simulink library "AEMS_Standard_Library"  (R2016b)
(part 11 of 39)

      settings: AttributesFormatString=%<MaskType>  RTWSystemCode=Nonreusable function  RTWFcnNameOpts=User specified
      mask Help:
      | eval('path_lib=fileparts(which(''AEMS_Standard_Library''));');
      | mskblk=get_param(gcbh,'MaskType');
      | doc_path = [path_lib '\Help\',mskblk,'.pdf'];
      | eval('open(doc_path)');
  AEMS_SUPPLIER_CALL_SEPA_MIN_LPOS : Subsystem  Tag=[LIB]  TreatAsAtomicUnit=on  RTWFcnName=SUPPLIER_CALL_Sepa_min_lpos  mask(AEMS_SUPPLIER_CALL_SEPA_MIN_LPOS){}
      mask help: Minimal separation time between 2 injection, depending on rail pressure and on fuel mass for open and close delays.
      mask init:
      | Thisblk = gcb;
      | model_type_pos = strsplit(Thisblk,'/');%to split all the layer paths in order to get the runnable path
      | runnable_path = [bdroot '/' model_type_pos{2}];%to get the runnable or AIPCALL path
      | trg_port_name = get_param(find_system(runnable_path,'BlockType','TriggerPort'),'Name');%to get the function call trigger name
      | TaskRate = '';%the raster suffix is stored in the parameter 
      | 
      | if ~isempty(trg_port_name)
      |     trg_port_name_spltd = strsplit(trg_port_name{1},'_');%splitting is done in order to get the raster and its type(Sched or Event)
      |     
      |     % checking for rasters of type Sched or Event especially occuring in
      |     % runnables
      |     if ~isempty(regexp(trg_port_name_spltd{1},'^Sched|^Event','once')) 
      |         TaskRate = ['_' regexprep(trg_port_name_spltd{1},'Sched|Event','','once')];
      |         
      |     %checking if the raster is dcmcb and this is applicable only for
      |     %APICALL
      |     elseif ~isempty(regexp([trg_port_name_spltd{1} '_' trg_port_name_spltd{2} '_' ],'^DataServices_DCM_|^RoutineServices_DCM_','once'))||...
      |             ~isempty(regexp(trg_port_name_spltd{1},'^Dcm$','once'))
      |         TaskRate = '_dcmcb';
      |         
      |     %checking if this block is used under the function call trigger
      |     %starting with "Com" and then giving an error message
      |     %this is applicable only for APICALL
      |     elseif ~isempty(regexp(trg_port_name_spltd{1},'^Com$','once'))
      |         msg = sprintf(['\n','The Supplier call block "' Thisblk '" should not be present within APICALLs having function call trigger as "Com"']);
      |         errordlg(msg);
      |         return;
      |     end
      | end
      | 
      | DataName = ['Supplier_Call_Sepa_Po_Lpost' TaskRate];%the variable name that should be given to DataStoreRead block 
      | set_param([Thisblk '/Data Store Read'],'DataStoreName',DataName);%Setting the DataStoreName of DataStoreRead block
      | 
      | %other settings done to this variable name
      | structVxx=Simulink.Signal;
      | structVxx.Dimensions=1;
      | structVxx.DimensionsMode='Fixed';
      | structVxx.DataType='single';
      | structVxx.Complexity='real';
      | structVxx.SamplingMode='Sample based';
      | structVxx.SampleTime=-1;
      | assignin('base',DataName,structVxx);
      settings: AttributesFormatString=%<MaskType>  RTWSystemCode=Nonreusable function  RTWFcnNameOpts=User specified
      mask Help:
      | eval('path_lib=fileparts(which(''AEMS_Standard_Library''));');
      | mskblk=get_param(gcbh,'MaskType');
      | doc_path = [path_lib '\Help\',mskblk,'.pdf'];
      | eval('open(doc_path)');
  AEMS_SUPPLIER_CALL_SEPA_MIN_LPOS2_2SL : Subsystem  Tag=[LIB]  TreatAsAtomicUnit=on  RTWFcnName=SUPPLIER_CALL_Sepa_min_lpos2_2sl  mask(AEMS_SUPPLIER_CALL_SEPA_MIN_LPOS2_2SL){}
      mask help: Minimal separation time between 2 injection, depending on rail pressure and on fuel mass for open and close delays.
      mask init:
      | Thisblk = gcb;
      | model_type_pos = strsplit(Thisblk,'/');%to split all the layer paths in order to get the runnable path
      | runnable_path = [bdroot '/' model_type_pos{2}];%to get the runnable or AIPCALL path
      | trg_port_name = get_param(find_system(runnable_path,'BlockType','TriggerPort'),'Name');%to get the function call trigger name
      | TaskRate = '';%the raster suffix is stored in the parameter 
      | 
      | if ~isempty(trg_port_name)
      |     trg_port_name_spltd = strsplit(trg_port_name{1},'_');%splitting is done in order to get the raster and its type(Sched or Event)
      |     
      |     % checking for rasters of type Sched or Event especially occuring in
      |     % runnables
      |     if ~isempty(regexp(trg_port_name_spltd{1},'^Sched|^Event','once')) 
      |         TaskRate = ['_' regexprep(trg_port_name_spltd{1},'Sched|Event','','once')];
      |         
      |     %checking if the raster is dcmcb and this is applicable only for
      |     %APICALL
      |     elseif ~isempty(regexp([trg_port_name_spltd{1} '_' trg_port_name_spltd{2} '_' ],'^DataServices_DCM_|^RoutineServices_DCM_','once'))||...
      |             ~isempty(regexp(trg_port_name_spltd{1},'^Dcm$','once'))
      |         TaskRate = '_dcmcb';
      |         
      |     %checking if this block is used under the function call trigger
      |     %starting with "Com" and then giving an error message
      |     %this is applicable only for APICALL
      |     elseif ~isempty(regexp(trg_port_name_spltd{1},'^Com$','once'))
      |         msg = sprintf(['\n','The Supplier call block "' Thisblk '" should not be present within APICALLs having function call trigger as "Com"']);
      |         errordlg(msg);
      |         return;
      |     end
      | end
      | 
      | DataName = ['Supplier_Call_Sepa_Lpost1_Lpost2' TaskRate];%the variable name that should be given to DataStoreRead block 
      | set_param([Thisblk '/Data Store Read'],'DataStoreName',DataName);%Setting the DataStoreName of DataStoreRead block
      | 
      | %other settings done to this variable name
      | structVxx=Simulink.Signal;
      | structVxx.Dimensions=1;
      | structVxx.DimensionsMode='Fixed';
      | structVxx.DataType='single';
      | structVxx.Complexity='real';
      | structVxx.SamplingMode='Sample based';
      | structVxx.SampleTime=-1;
      | assignin('base',DataName,structVxx);
      settings: AttributesFormatString=%<MaskType>  RTWSystemCode=Nonreusable function  RTWFcnNameOpts=User specified
      mask Help:
      | eval('path_lib=fileparts(which(''AEMS_Standard_Library''));');
      | mskblk=get_param(gcbh,'MaskType');
      | doc_path = [path_lib '\Help\',mskblk,'.pdf'];
      | eval('open(doc_path)');
  AEMS_SUPPLIER_CALL_SEPA_MIN_LPOS2_3SL : Subsystem  Tag=[LIB]  TreatAsAtomicUnit=on  RTWFcnName=SUPPLIER_CALL_Sepa_min_lpos2_3sl  mask(AEMS_SUPPLIER_CALL_SEPA_MIN_LPOS2_3SL){}
      mask help: Minimal separation time between 2 injection, depending on rail pressure and on fuel mass for open and close delays.
      mask init: same as AEMS_Standard_Library/SPECIFIC/AEMS_SUPPLIER_CALL_SEPA_MIN_LPOS2_2SL
      settings: AttributesFormatString=%<MaskType>  RTWSystemCode=Nonreusable function  RTWFcnNameOpts=User specified
      mask Help:
      | eval('path_lib=fileparts(which(''AEMS_Standard_Library''));');
      | mskblk=get_param(gcbh,'MaskType');
      | doc_path = [path_lib '\Help\',mskblk,'.pdf'];
      | eval('open(doc_path)');
  AEMS_SUPPLIER_CALL_SEPA_MIN_LPOS2_4SL : Subsystem  Tag=[LIB]  TreatAsAtomicUnit=on  RTWFcnName=SUPPLIER_CALL_Sepa_min_lpos2_4sl  mask(AEMS_SUPPLIER_CALL_SEPA_MIN_LPOS2_4SL){}
      mask help: Minimal separation time between 2 injection, depending on rail pressure and on fuel mass for open and close delays.
      mask init: same as AEMS_Standard_Library/SPECIFIC/AEMS_SUPPLIER_CALL_SEPA_MIN_LPOS2_2SL
      settings: AttributesFormatString=%<MaskType>  RTWSystemCode=Nonreusable function  RTWFcnNameOpts=User specified
      mask Help:
      | eval('path_lib=fileparts(which(''AEMS_Standard_Library''));');
      | mskblk=get_param(gcbh,'MaskType');
      | doc_path = [path_lib '\Help\',mskblk,'.pdf'];
      | eval('open(doc_path)');
  AEMS_SUPPLIER_CALL_SEPA_MIN_LPOS3_3SL : Subsystem  Tag=[LIB]  TreatAsAtomicUnit=on  RTWFcnName=SUPPLIER_CALL_Sepa_min_lpos3_3sl  mask(AEMS_SUPPLIER_CALL_SEPA_MIN_LPOS3_3SL){}
      mask help: Minimal separation time between 2 injection, depending on rail pressure and on fuel mass for open and close delays.
      mask init: same as AEMS_Standard_Library/SPECIFIC/AEMS_SUPPLIER_CALL_SEPA_MIN_LPOS2_2SL
      settings: AttributesFormatString=%<MaskType>  RTWSystemCode=Nonreusable function  RTWFcnNameOpts=User specified
      mask Help:
      | eval('path_lib=fileparts(which(''AEMS_Standard_Library''));');
      | mskblk=get_param(gcbh,'MaskType');
      | doc_path = [path_lib '\Help\',mskblk,'.pdf'];
      | eval('open(doc_path)');
  AEMS_SUPPLIER_CALL_SEPA_MIN_LPOS3_4SL : Subsystem  Tag=[LIB]  TreatAsAtomicUnit=on  RTWFcnName=SUPPLIER_CALL_Sepa_min_lpos3_4sl  mask(AEMS_SUPPLIER_CALL_SEPA_MIN_LPOS3_4SL){}
      mask help: Minimal separation time between 2 injection, depending on rail pressure and on fuel mass for open and close delays.
      mask init: same as AEMS_Standard_Library/SPECIFIC/AEMS_SUPPLIER_CALL_SEPA_MIN_LPOS2_2SL
      settings: AttributesFormatString=%<MaskType>  RTWSystemCode=Nonreusable function  RTWFcnNameOpts=User specified
      mask Help:
      | eval('path_lib=fileparts(which(''AEMS_Standard_Library''));');
      | mskblk=get_param(gcbh,'MaskType');
      | doc_path = [path_lib '\Help\',mskblk,'.pdf'];
      | eval('open(doc_path)');
  AEMS_SUPPLIER_CALL_SEPA_MIN_LPOS4_4SL : Subsystem  Tag=[LIB]  TreatAsAtomicUnit=on  RTWFcnName=SUPPLIER_CALL_Sepa_min_lpos4_4sl  mask(AEMS_SUPPLIER_CALL_SEPA_MIN_LPOS4_4SL){}
      mask help: Minimal separation time between 2 injection, depending on rail pressure and on fuel mass for open and close delays.
      mask init: same as AEMS_Standard_Library/SPECIFIC/AEMS_SUPPLIER_CALL_SEPA_MIN_LPOS2_2SL
      settings: AttributesFormatString=%<MaskType>  RTWSystemCode=Nonreusable function  RTWFcnNameOpts=User specified
      mask Help:
      | eval('path_lib=fileparts(which(''AEMS_Standard_Library''));');
      | mskblk=get_param(gcbh,'MaskType');
      | doc_path = [path_lib '\Help\',mskblk,'.pdf'];
      | eval('open(doc_path)');
  AEMS_SUPPLIER_CALL_SEPA_MIN_NXT_CYL : Subsystem  Tag=[LIB]  TreatAsAtomicUnit=on  RTWFcnName=SUPPLIER_CALL_Sepa_min_nxt_cyl  mask(AEMS_SUPPLIER_CALL_SEPA_MIN_NXT_CYL){}
      mask help: Minimal separation time between 2 injection, depending on rail pressure and on fuel mass for open and close delays.
      mask init:
      | Thisblk = gcb;
      | model_type_pos = strsplit(Thisblk,'/');%to split all the layer paths in order to get the runnable path
      | runnable_path = [bdroot '/' model_type_pos{2}];%to get the runnable or AIPCALL path
      | trg_port_name = get_param(find_system(runnable_path,'BlockType','TriggerPort'),'Name');%to get the function call trigger name
      | TaskRate = '';%the raster suffix is stored in the parameter 
      | 
      | if ~isempty(trg_port_name)
      |     trg_port_name_spltd = strsplit(trg_port_name{1},'_');%splitting is done in order to get the raster and its type(Sched or Event)
      |     
      |     % checking for rasters of type Sched or Event especially occuring in
      |     % runnables
      |     if ~isempty(regexp(trg_port_name_spltd{1},'^Sched|^Event','once')) 
      |         TaskRate = ['_' regexprep(trg_port_name_spltd{1},'Sched|Event','','once')];
      |         
      |     %checking if the raster is dcmcb and this is applicable only for
      |     %APICALL
      |     elseif ~isempty(regexp([trg_port_name_spltd{1} '_' trg_port_name_spltd{2} '_' ],'^DataServices_DCM_|^RoutineServices_DCM_','once'))||...
      |             ~isempty(regexp(trg_port_name_spltd{1},'^Dcm$','once'))
      |         TaskRate = '_dcmcb';
      |         
      |     %checking if this block is used under the function call trigger
      |     %starting with "Com" and then giving an error message
      |     %this is applicable only for APICALL
      |     elseif ~isempty(regexp(trg_port_name_spltd{1},'^Com$','once'))
      |         msg = sprintf(['\n','The Supplier call block "' Thisblk '" should not be present within APICALLs having function call trigger as "Com"']);
      |         errordlg(msg);
      |         return;
      |     end
      | end
      | 
      | DataName = ['Supplier_Call_Sepa_Lpost_Pinj' TaskRate];%the variable name that should be given to DataStoreRead block 
      | set_param([Thisblk '/Data Store Read'],'DataStoreName',DataName);%Setting the DataStoreName of DataStoreRead block
      | 
      | %other settings done to this variable name
      | structVxx=Simulink.Signal;
      | structVxx.Dimensions=1;
      | structVxx.DimensionsMode='Fixed';
      | structVxx.DataType='single';
      | structVxx.Complexity='real';
      | structVxx.SamplingMode='Sample based';
      | structVxx.SampleTime=-1;
      | assignin('base',DataName,structVxx);
      settings: AttributesFormatString=%<MaskType>  RTWSystemCode=Nonreusable function  RTWFcnNameOpts=User specified
      mask Help:
      | eval('path_lib=fileparts(which(''AEMS_Standard_Library''));');
      | mskblk=get_param(gcbh,'MaskType');
      | doc_path = [path_lib '\Help\',mskblk,'.pdf'];
      | eval('open(doc_path)');
  AEMS_SUPPLIER_CALL_SEPA_MIN_NXT_CYL_LPOST2 : Subsystem  Tag=[LIB]  TreatAsAtomicUnit=on  RTWFcnName=SUPPLIER_CALL_Sepa_min_nxt_cyl_lpost2  mask(AEMS_SUPPLIER_CALL_SEPA_MIN_NXT_CYL_LPOST2){}
      mask help: Minimal separation time between 2 injection, depending on rail pressure and on fuel mass for open and close delays.
      mask init: same as AEMS_Standard_Library/SPECIFIC/AEMS_SUPPLIER_CALL_SEPA_MIN_NXT_CYL
      settings: AttributesFormatString=%<MaskType>  RTWSystemCode=Nonreusable function  RTWFcnNameOpts=User specified
      mask Help:
      | eval('path_lib=fileparts(which(''AEMS_Standard_Library''));');
      | mskblk=get_param(gcbh,'MaskType');
      | doc_path = [path_lib '\Help\',mskblk,'.pdf'];
      | eval('open(doc_path)');
  AEMS_SUPPLIER_CALL_SEPA_MIN_NXT_CYL_LPOST3 : Subsystem  Tag=[LIB]  TreatAsAtomicUnit=on  RTWFcnName=SUPPLIER_CALL_Sepa_min_nxt_cyl_lpost3  mask(AEMS_SUPPLIER_CALL_SEPA_MIN_NXT_CYL_LPOST3){}
      mask help: Minimal separation time between 2 injection, depending on rail pressure and on fuel mass for open and close delays.
      mask init: same as AEMS_Standard_Library/SPECIFIC/AEMS_SUPPLIER_CALL_SEPA_MIN_NXT_CYL
      settings: AttributesFormatString=%<MaskType>  RTWSystemCode=Nonreusable function  RTWFcnNameOpts=User specified
      mask Help:
      | eval('path_lib=fileparts(which(''AEMS_Standard_Library''));');
      | mskblk=get_param(gcbh,'MaskType');
      | doc_path = [path_lib '\Help\',mskblk,'.pdf'];
      | eval('open(doc_path)');
  AEMS_SUPPLIER_CALL_SEPA_MIN_NXT_CYL_LPOST4 : Subsystem  Tag=[LIB]  TreatAsAtomicUnit=on  RTWFcnName=SUPPLIER_CALL_Sepa_min_nxt_cyl_lpost4  mask(AEMS_SUPPLIER_CALL_SEPA_MIN_NXT_CYL_LPOST4){}
      mask help: Minimal separation time between 2 injection, depending on rail pressure and on fuel mass for open and close delays.
      mask init: same as AEMS_Standard_Library/SPECIFIC/AEMS_SUPPLIER_CALL_SEPA_MIN_NXT_CYL
      settings: AttributesFormatString=%<MaskType>  RTWSystemCode=Nonreusable function  RTWFcnNameOpts=User specified
      mask Help:
      | eval('path_lib=fileparts(which(''AEMS_Standard_Library''));');
      | mskblk=get_param(gcbh,'MaskType');
      | doc_path = [path_lib '\Help\',mskblk,'.pdf'];
      | eval('open(doc_path)');
  AEMS_SUPPLIER_CALL_SEPA_MIN_PINJ1 : Subsystem  Tag=[LIB]  TreatAsAtomicUnit=on  RTWFcnName=SUPPLIER_CALL_Sepa_min_pinj1  mask(AEMS_SUPPLIER_CALL_SEPA_MIN_PINJ1){}
      mask help: Minimal separation time between 2 injection, depending on rail pressure and on fuel mass for open and close delays.
      mask init:
      | Thisblk = gcb;
      | model_type_pos = strsplit(Thisblk,'/');%to split all the layer paths in order to get the runnable path
      | runnable_path = [bdroot '/' model_type_pos{2}];%to get the runnable or AIPCALL path
      | trg_port_name = get_param(find_system(runnable_path,'BlockType','TriggerPort'),'Name');%to get the function call trigger name
      | TaskRate = '';%the raster suffix is stored in the parameter 
      | 
      | if ~isempty(trg_port_name)
      |     trg_port_name_spltd = strsplit(trg_port_name{1},'_');%splitting is done in order to get the raster and its type(Sched or Event)
      |     
      |     % checking for rasters of type Sched or Event especially occuring in
      |     % runnables
      |     if ~isempty(regexp(trg_port_name_spltd{1},'^Sched|^Event','once')) 
      |         TaskRate = ['_' regexprep(trg_port_name_spltd{1},'Sched|Event','','once')];
      |         
      |     %checking if the raster is dcmcb and this is applicable only for
      |     %APICALL
      |     elseif ~isempty(regexp([trg_port_name_spltd{1} '_' trg_port_name_spltd{2} '_' ],'^DataServices_DCM_|^RoutineServices_DCM_','once'))||...
      |             ~isempty(regexp(trg_port_name_spltd{1},'^Dcm$','once'))
      |         TaskRate = '_dcmcb';
      |         
      |     %checking if this block is used under the function call trigger
      |     %starting with "Com" and then giving an error message
      |     %this is applicable only for APICALL
      |     elseif ~isempty(regexp(trg_port_name_spltd{1},'^Com$','once'))
      |         msg = sprintf(['\n','The Supplier call block "' Thisblk '" should not be present within APICALLs having function call trigger as "Com"']);
      |         errordlg(msg);
      |         return;
      |     end
      | end
      | 
      | DataName = ['Supplier_Call_Sepa_P1_P2' TaskRate];%the variable name that should be given to DataStoreRead block 
      | set_param([Thisblk '/Data Store Read'],'DataStoreName',DataName);%Setting the DataStoreName of DataStoreRead block
      | 
      | %other settings done to this variable name
      | structVxx=Simulink.Signal;
      | structVxx.Dimensions=1;
      | structVxx.DimensionsMode='Fixed';
      | structVxx.DataType='single';
      | structVxx.Complexity='real';
      | structVxx.SamplingMode='Sample based';
      | structVxx.SampleTime=-1;
      | assignin('base',DataName,structVxx);
      settings: AttributesFormatString=%<MaskType>  RTWSystemCode=Nonreusable function  RTWFcnNameOpts=User specified
      mask Help:
      | eval('path_lib=fileparts(which(''AEMS_Standard_Library''));');
      | mskblk=get_param(gcbh,'MaskType');
      | doc_path = [path_lib '\Help\',mskblk,'.pdf'];
      | eval('open(doc_path)');
  AEMS_SUPPLIER_CALL_SEPA_MIN_PINJ2 : Subsystem  Tag=[LIB]  TreatAsAtomicUnit=on  RTWFcnName=SUPPLIER_CALL_Sepa_min_pinj2  mask(AEMS_SUPPLIER_CALL_SEPA_MIN_PINJ2){}
      mask help: Minimal separation time between 2 injection, depending on rail pressure and on fuel mass for open and close delays.
      mask init:
      | Thisblk = gcb;
      | model_type_pos = strsplit(Thisblk,'/');%to split all the layer paths in order to get the runnable path
      | runnable_path = [bdroot '/' model_type_pos{2}];%to get the runnable or AIPCALL path
      | trg_port_name = get_param(find_system(runnable_path,'BlockType','TriggerPort'),'Name');%to get the function call trigger name
      | TaskRate = '';%the raster suffix is stored in the parameter 
      | 
      | if ~isempty(trg_port_name)
      |     trg_port_name_spltd = strsplit(trg_port_name{1},'_');%splitting is done in order to get the raster and its type(Sched or Event)
      |     
      |     % checking for rasters of type Sched or Event especially occuring in
      |     % runnables
      |     if ~isempty(regexp(trg_port_name_spltd{1},'^Sched|^Event','once')) 
      |         TaskRate = ['_' regexprep(trg_port_name_spltd{1},'Sched|Event','','once')];
      |         
      |     %checking if the raster is dcmcb and this is applicable only for
      |     %APICALL
      |     elseif ~isempty(regexp([trg_port_name_spltd{1} '_' trg_port_name_spltd{2} '_' ],'^DataServices_DCM_|^RoutineServices_DCM_','once'))||...
      |             ~isempty(regexp(trg_port_name_spltd{1},'^Dcm$','once'))
      |         TaskRate = '_dcmcb';
      |         
      |     %checking if this block is used under the function call trigger
      |     %starting with "Com" and then giving an error message
      |     %this is applicable only for APICALL
      |     elseif ~isempty(regexp(trg_port_name_spltd{1},'^Com$','once'))
      |         msg = sprintf(['\n','The Supplier call block "' Thisblk '" should not be present within APICALLs having function call trigger as "Com"']);
      |         errordlg(msg);
      |         return;
      |     end
      | end
      | 
      | DataName = ['Supplier_Call_Sepa_P2_P3' TaskRate];%the variable name that should be given to DataStoreRead block 
      | set_param([Thisblk '/Data Store Read'],'DataStoreName',DataName);%Setting the DataStoreName of DataStoreRead block
      | 
      | %other settings done to this variable name
      | structVxx=Simulink.Signal;
      | structVxx.Dimensions=1;
      | structVxx.DimensionsMode='Fixed';
      | structVxx.DataType='single';
      | structVxx.Complexity='real';
      | structVxx.SamplingMode='Sample based';
      | structVxx.SampleTime=-1;
      | assignin('base',DataName,structVxx);
      settings: AttributesFormatString=%<MaskType>  RTWSystemCode=Nonreusable function  RTWFcnNameOpts=User specified
      mask Help:
      | eval('path_lib=fileparts(which(''AEMS_Standard_Library''));');
      | mskblk=get_param(gcbh,'MaskType');
      | doc_path = [path_lib '\Help\',mskblk,'.pdf'];
      | eval('open(doc_path)');
  AEMS_SUPPLIER_CALL_SEPA_MIN_PINJ3 : Subsystem  Tag=[LIB]  TreatAsAtomicUnit=on  RTWFcnName=SUPPLIER_CALL_Sepa_min_pinj3  mask(AEMS_SUPPLIER_CALL_SEPA_MIN_PINJ3){}
      mask help: Minimal separation time between 2 injection, depending on rail pressure and on fuel mass for open and close delays.
      mask init:
      | Thisblk = gcb;
      | model_type_pos = strsplit(Thisblk,'/');%to split all the layer paths in order to get the runnable path
      | runnable_path = [bdroot '/' model_type_pos{2}];%to get the runnable or AIPCALL path
      | trg_port_name = get_param(find_system(runnable_path,'BlockType','TriggerPort'),'Name');%to get the function call trigger name
      | TaskRate = '';%the raster suffix is stored in the parameter 
      | 
      | if ~isempty(trg_port_name)
      |     trg_port_name_spltd = strsplit(trg_port_name{1},'_');%splitting is done in order to get the raster and its type(Sched or Event)
      |     
      |     % checking for rasters of type Sched or Event especially occuring in
      |     % runnables
      |     if ~isempty(regexp(trg_port_name_spltd{1},'^Sched|^Event','once')) 
      |         TaskRate = ['_' regexprep(trg_port_name_spltd{1},'Sched|Event','','once')];
      |         
      |     %checking if the raster is dcmcb and this is applicable only for
      |     %APICALL
      |     elseif ~isempty(regexp([trg_port_name_spltd{1} '_' trg_port_name_spltd{2} '_' ],'^DataServices_DCM_|^RoutineServices_DCM_','once'))||...
      |             ~isempty(regexp(trg_port_name_spltd{1},'^Dcm$','once'))
      |         TaskRate = '_dcmcb';
      |         
      |     %checking if this block is used under the function call trigger
      |     %starting with "Com" and then giving an error message
      |     %this is applicable only for APICALL
      |     elseif ~isempty(regexp(trg_port_name_spltd{1},'^Com$','once'))
      |         msg = sprintf(['\n','The Supplier call block "' Thisblk '" should not be present within APICALLs having function call trigger as "Com"']);
      |         errordlg(msg);
      |         return;
      |     end
      | end
      | 
      | DataName = ['Supplier_Call_Sepa_P3_P4' TaskRate];%the variable name that should be given to DataStoreRead block 
      | set_param([Thisblk '/Data Store Read'],'DataStoreName',DataName);%Setting the DataStoreName of DataStoreRead block
      | 
      | %other settings done to this variable name
      | structVxx=Simulink.Signal;
      | structVxx.Dimensions=1;
      | structVxx.DimensionsMode='Fixed';
      | structVxx.DataType='single';
      | structVxx.Complexity='real';
      | structVxx.SamplingMode='Sample based';
      | structVxx.SampleTime=-1;
      | assignin('base',DataName,structVxx);
      settings: AttributesFormatString=%<MaskType>  RTWSystemCode=Nonreusable function  RTWFcnNameOpts=User specified
      mask Help:
      | eval('path_lib=fileparts(which(''AEMS_Standard_Library''));');
      | mskblk=get_param(gcbh,'MaskType');
      | doc_path = [path_lib '\Help\',mskblk,'.pdf'];
      | eval('open(doc_path)');
  AEMS_SUPPLIER_CALL_SEPA_MIN_PINJ4 : Subsystem  Tag=[LIB]  TreatAsAtomicUnit=on  RTWFcnName=SUPPLIER_CALL_Sepa_min_pinj4  mask(AEMS_SUPPLIER_CALL_SEPA_MIN_PINJ4){}
      mask help: Minimal separation time between 2 injection, depending on rail pressure and on fuel mass for open and close delays.
      mask init:
      | Thisblk = gcb;
      | model_type_pos = strsplit(Thisblk,'/');%to split all the layer paths in order to get the runnable path
      | runnable_path = [bdroot '/' model_type_pos{2}];%to get the runnable or AIPCALL path
      | trg_port_name = get_param(find_system(runnable_path,'BlockType','TriggerPort'),'Name');%to get the function call trigger name
      | TaskRate = '';%the raster suffix is stored in the parameter 
      | 
      | if ~isempty(trg_port_name)
      |     trg_port_name_spltd = strsplit(trg_port_name{1},'_');%splitting is done in order to get the raster and its type(Sched or Event)
      |     
      |     % checking for rasters of type Sched or Event especially occuring in
      |     % runnables
      |     if ~isempty(regexp(trg_port_name_spltd{1},'^Sched|^Event','once')) 
      |         TaskRate = ['_' regexprep(trg_port_name_spltd{1},'Sched|Event','','once')];
      |         
      |     %checking if the raster is dcmcb and this is applicable only for
      |     %APICALL
      |     elseif ~isempty(regexp([trg_port_name_spltd{1} '_' trg_port_name_spltd{2} '_' ],'^DataServices_DCM_|^RoutineServices_DCM_','once'))||...
      |             ~isempty(regexp(trg_port_name_spltd{1},'^Dcm$','once'))
      |         TaskRate = '_dcmcb';
      |         
      |     %checking if this block is used under the function call trigger
      |     %starting with "Com" and then giving an error message
      |     %this is applicable only for APICALL
      |     elseif ~isempty(regexp(trg_port_name_spltd{1},'^Com$','once'))
      |         msg = sprintf(['\n','The Supplier call block "' Thisblk '" should not be present within APICALLs having function call trigger as "Com"']);
      |         errordlg(msg);
      |         return;
      |     end
      | end
      | 
      | DataName = ['Supplier_Call_Sepa_Pinj_Main' TaskRate];%the variable name that should be given to DataStoreRead block 
      | set_param([Thisblk '/Data Store Read'],'DataStoreName',DataName);%Setting the DataStoreName of DataStoreRead block
      | 
      | %other settings done to this variable name
      | structVxx=Simulink.Signal;
      | structVxx.Dimensions=1;
      | structVxx.DimensionsMode='Fixed';
      | structVxx.DataType='single';
      | structVxx.Complexity='real';
      | structVxx.SamplingMode='Sample based';
      | structVxx.SampleTime=-1;
      | assignin('base',DataName,structVxx);
      settings: AttributesFormatString=%<MaskType>  RTWSystemCode=Nonreusable function  RTWFcnNameOpts=User specified
      mask Help:
      | eval('path_lib=fileparts(which(''AEMS_Standard_Library''));');
      | mskblk=get_param(gcbh,'MaskType');
      | doc_path = [path_lib '\Help\',mskblk,'.pdf'];
      | eval('open(doc_path)');
  AEMS_SUPPLIER_CALL_SEPA_MIN_POST : Subsystem  Tag=[LIB]  TreatAsAtomicUnit=on  RTWFcnName=SUPPLIER_CALL_Sepa_min_post  mask(AEMS_SUPPLIER_CALL_SEPA_MIN_POST){}
      mask help: Minimal separation time between 2 injection, depending on rail pressure and on fuel mass for open and close delays.
      mask init:
      | Thisblk = gcb;
      | model_type_pos = strsplit(Thisblk,'/');%to split all the layer paths in order to get the runnable path
      | runnable_path = [bdroot '/' model_type_pos{2}];%to get the runnable or AIPCALL path
      | trg_port_name = get_param(find_system(runnable_path,'BlockType','TriggerPort'),'Name');%to get the function call trigger name
      | TaskRate = '';%the raster suffix is stored in the parameter 
      | 
      | if ~isempty(trg_port_name)
      |     trg_port_name_spltd = strsplit(trg_port_name{1},'_');%splitting is done in order to get the raster and its type(Sched or Event)
      |     
      |     % checking for rasters of type Sched or Event especially occuring in
      |     % runnables
      |     if ~isempty(regexp(trg_port_name_spltd{1},'^Sched|^Event','once')) 
      |         TaskRate = ['_' regexprep(trg_port_name_spltd{1},'Sched|Event','','once')];
      |         
      |     %checking if the raster is dcmcb and this is applicable only for
      |     %APICALL
      |     elseif ~isempty(regexp([trg_port_name_spltd{1} '_' trg_port_name_spltd{2} '_' ],'^DataServices_DCM_|^RoutineServices_DCM_','once'))||...
      |             ~isempty(regexp(trg_port_name_spltd{1},'^Dcm$','once'))
      |         TaskRate = '_dcmcb';
      |         
      |     %checking if this block is used under the function call trigger
      |     %starting with "Com" and then giving an error message
      |     %this is applicable only for APICALL
      |     elseif ~isempty(regexp(trg_port_name_spltd{1},'^Com$','once'))
      |         msg = sprintf(['\n','The Supplier call block "' Thisblk '" should not be present within APICALLs having function call trigger as "Com"']);
      |         errordlg(msg);
      |         return;
      |     end
      | end
      | 
      | DataName = ['Supplier_Call_Sepa_Main_Af_Po' TaskRate];%the variable name that should be given to DataStoreRead block 
      | set_param([Thisblk '/Data Store Read'],'DataStoreName',DataName);%Setting the DataStoreName of DataStoreRead block
      | 
      | %other settings done to this variable name
      | structVxx=Simulink.Signal;
      | structVxx.Dimensions=1;
      | structVxx.DimensionsMode='Fixed';
      | structVxx.DataType='single';
      | structVxx.Complexity='real';
      | structVxx.SamplingMode='Sample based';
      | structVxx.SampleTime=-1;
      | assignin('base',DataName,structVxx);
      settings: AttributesFormatString=%<MaskType>  RTWSystemCode=Nonreusable function  RTWFcnNameOpts=User specified
      mask Help:
      | eval('path_lib=fileparts(which(''AEMS_Standard_Library''));');
      | mskblk=get_param(gcbh,'MaskType');
      | doc_path = [path_lib '\Help\',mskblk,'.pdf'];
      | eval('open(doc_path)');
  AEMS_SUPPLIER_CALL_SEPERATION_MIN_TIME : Subsystem  Tag=[LIB]  TreatAsAtomicUnit=on  RTWFcnName=SUPPLIER_CALL_Sepa_min_post1  mask(AEMS_SUPPLIER_CALL_SEPERATION_MIN_TIME){Outportname=Vxx_fms_sep_min_post2_3sl, Suppliercallname=SUPPLIER_CALL_Sepa_min_post2, Splitnum=3}
      mask prompts: Outportname "Outport Name"; Suppliercallname "Supplier call Name"; Splitnum "Split"
      mask help:
      | Minimal separation time between 2 injection, depending on rail pressure
      | and on fuel mass for open and close delays.
      |
      | Each block will be translated into code C by this way:
      | Output=Supplier call API Name(Splitnum);
      | Example for Supplier_Call_Sepa_min_post1, corresponding output variable is
      | Vxx_fms_sep_min_post1= Supplier_Call_Sepa_min_post1(1);
      mask init:
      | ThisBlk = gcb;
      | OutPorts            =   {'Vxx_fms_sep_min_post1','Vxx_fms_sep_min_post1_2sl','Vxx_fms_sep_min_post1_3sl','Vxx_fms_sep_min_post2_2sl','Vxx_fms_sep_min_post2_3sl','Vxx_fms_sep_min_post3_3sl'};
      | 
      | Supplier_Calls      =   {'SUPPLIER_CALL_Sepa_min_post1','SUPPLIER_CALL_Sepa_min_post1','SUPPLIER_CALL_Sepa_min_post1','SUPPLIER_CALL_Sepa_min_post2','SUPPLIER_CALL_Sepa_min_post2','SUPPLIER_CALL_Sepa_min_post3'};
      | 
      | Data_Names          =   {'Supplier_Call_Sepa_min_post1','Supplier_Call_Sepa_min_post1','Supplier_Call_Sepa_min_post1','Supplier_Call_Sepa_min_post2','Supplier_Call_Sepa_min_post2','Supplier_Call_Sepa_min_post3'};                      
      |                       
      |                       
      | Splits              =   {'1','2','3','2','3','3'};
      | 
      | model_type_pos = strsplit(ThisBlk,'/');
      | runnable_path = [bdroot '/' model_type_pos{2}];%to get the runnable or APICALL path
      | trg_port_name = get_param(find_system(runnable_path,'BlockType','TriggerPort'),'Name');%to get the function call trigger name
      | TaskRate = '';
      | if ~isempty(trg_port_name)
      |     trg_port_name_spltd = strsplit(trg_port_name{1},'_');
      |     if ~isempty(regexp(trg_port_name_spltd{1},'^Sched|^Event','once'))
      |         TaskRate = ['_' regexprep(trg_port_name_spltd{1},'Sched|Event','','once')];
      |     elseif ~isempty(regexp([trg_port_name_spltd{1} '_' trg_port_name_spltd{2} '_' ],'^DataServices_DCM_|^RoutineServices_DCM_','once'))||...
      |             ~isempty(regexp(trg_port_name_spltd{1},'^Dcm$','once'))
      |         TaskRate = '_dcmcb';
      |     elseif ~isempty(regexp(trg_port_name_spltd{1},'^Com$','once'))
      |         msg = sprintf(['\n','The Supplier call block "' Thisblk '" should not be present within APICALLs having function call trigger as "Com"']);
      |         errordlg(msg);
      |         return;
      |     end
      | end
      | 
      | Idx_Of_Outportname = find(ismember(OutPorts,Outportname));
      | DataName = [Data_Names{Idx_Of_Outportname} TaskRate];
      | 
      | %set the  suppliername according to the Outport name.
      | set_param(ThisBlk,'Suppliercallname',Supplier_Calls{Idx_Of_Outportname});
      | set_param(ThisBlk,'Splitnum',Splits{Idx_Of_Outportname});
      | 
      | %Get the paths of the blks under this lib block.
      | Const_Blk = [ThisBlk,'/Splitnum'];%%path of "const block" inside this lib blk.
      | DSR_Blk   = [ThisBlk,'/Data_Store_Read'];%path of "Data store read block" inside this lib blk.
      | Outport_Blk = find_system(ThisBlk,'LookUnderMasks','all','FollowLinks','on','BlockType','Outport');
      | Outport_Blk = Outport_Blk{1};%I know this is d only outport blk.
      | 
      | %set the attributes of the blks under this lib block, based on teh Outportname chosen by d user.
      | set_param(Outport_Blk,'Name',Outportname);
      | set_param(DSR_Blk,'DataStoreName',DataName);
      | set_param(Const_Blk,'Value',Splits{Idx_Of_Outportname});
      | 
      | %To create a singal object in d base workspace.
      | EvalStr = ['exist(''',DataName,''',''var'')'];
      | structVxx=Simulink.Signal;
      | % structVxx=Simulink.Signal;
      | structVxx.Dimensions=1;
      | structVxx.DimensionsMode='Fixed';
      | structVxx.DataType='single';
      | structVxx.Complexity='real';
      | structVxx.SamplingMode='Sample based';
      | structVxx.SampleTime=-1;
      | isDefined= evalin('base',EvalStr);%This line checks whether the DataName exist in the base workspace.
      | if (isDefined==0)
      |     assignin('base',DataName,structVxx);
      | end
      settings: RTWSystemCode=Inline  RTWFcnNameOpts=User specified
      settings: AttributesFormatString=|
      | %<MaskType>
      | Supplier Call Name = %<Suppliercallname>
      | Outport Name = %<Outportname>\nSplit Number = %<Splitnum>
      mask Help:
      | eval('path_lib=fileparts(which(''AEMS_Standard_Library''));');
      | mskblk=get_param(gcbh,'MaskType');
      | doc_path = [path_lib '\Help\',mskblk,'.pdf'];
      | eval('open(doc_path)');
      mask TypeOptions Outportname: Vxx_fms_sep_min_post1 | Vxx_fms_sep_min_post1_2sl | Vxx_fms_sep_min_post1_3sl | Vxx_fms_sep_min_post2_2sl | Vxx_fms_sep_min_post2_3sl | Vxx_fms_sep_min_post3_3sl
      mask Callback Outportname:
      | OutPorts            =   {'Vxx_fms_sep_min_post1','Vxx_fms_sep_min_post1_2sl','Vxx_fms_sep_min_post1_3sl','Vxx_fms_sep_min_post2_2sl','Vxx_fms_sep_min_post2_3sl','Vxx_fms_sep_min_post3_3sl'};
      | 
      | Supplier_Calls      =   {'SUPPLIER_CALL_Sepa_min_post1','SUPPLIER_CALL_Sepa_min_post1','SUPPLIER_CALL_Sepa_min_post1','SUPPLIER_CALL_Sepa_min_post2','SUPPLIER_CALL_Sepa_min_post2','SUPPLIER_CALL_Sepa_min_post3'};
      | 
      | Splits              =   {'1','2','3','2','3','3'};
      | 
      | Outportname = get_param(gcb,'Outportname');
      | 
      | Idx_Of_Outportname = find(ismember(OutPorts,Outportname));
      | %set the  suppliername according to the Outport name.
      | set_param(gcb,'Suppliercallname',Supplier_Calls{Idx_Of_Outportname});
      | set_param(gcb,'Splitnum',Splits{Idx_Of_Outportname});
      | cellfun(@clear,{'Idx_Of_Outportname','Outportname','OutPorts','Splits','Supplier_Calls'});
  AEMS_SUPPLIER_CALL_TI_MINI_OK_AFTR : Subsystem  Tag=[LIB]  TreatAsAtomicUnit=on  RTWFcnName=SUPPLIER_CALL_Ti_mini_ok_aftr  mask(AEMS_SUPPLIER_CALL_TI_MINI_OK_AFTR){}
      mask help:
      | Verify if the estimated fuel injection ti is over minimum possible ti.
      |
      | This block is to call Supplier call API.
      mask init:
      | Thisblk = gcb;
      | model_type_pos = strsplit(Thisblk,'/');%to split all the layer paths in order to get the runnable path
      | runnable_path = [bdroot '/' model_type_pos{2}];%to get the runnable or AIPCALL path
      | trg_port_name = get_param(find_system(runnable_path,'BlockType','TriggerPort'),'Name');%to get the function call trigger name
      | TaskRate = '';%the raster suffix is stored in the parameter 
      | 
      | if ~isempty(trg_port_name)
      |     trg_port_name_spltd = strsplit(trg_port_name{1},'_');%splitting is done in order to get the raster and its type(Sched or Event)
      |     
      |     % checking for rasters of type Sched or Event especially occuring in
      |     % runnables
      |     if ~isempty(regexp(trg_port_name_spltd{1},'^Sched|^Event','once')) 
      |         TaskRate = ['_' regexprep(trg_port_name_spltd{1},'Sched|Event','','once')];
      |         
      |     %checking if the raster is dcmcb and this is applicable only for
      |     %APICALL
      |     elseif ~isempty(regexp([trg_port_name_spltd{1} '_' trg_port_name_spltd{2} '_' ],'^DataServices_DCM_|^RoutineServices_DCM_','once'))||...
      |             ~isempty(regexp(trg_port_name_spltd{1},'^Dcm$','once'))
      |         TaskRate = '_dcmcb';
      |         
      |     %checking if this block is used under the function call trigger
      |     %starting with "Com" and then giving an error message
      |     %this is applicable only for APICALL
      |     elseif ~isempty(regexp(trg_port_name_spltd{1},'^Com$','once'))
      |         msg = sprintf(['\n','The Supplier call block "' Thisblk '" should not be present within APICALLs having function call trigger as "Com"']);
      |         errordlg(msg);
      |         return;
      |     end
      | end
      | 
      | DataName = ['Supplier_call_ti_mini_ok_aftr' TaskRate];%the variable name that should be given to DataStoreRead block 
      | set_param([Thisblk '/Data Store Read'],'DataStoreName',DataName);%Setting the DataStoreName of DataStoreRead block
      | 
      | %other settings done to this variable name
      | structVxx=Simulink.Signal;
      | structVxx.Dimensions=1;
      | structVxx.DimensionsMode='Fixed';
      | structVxx.DataType='boolean';
      | structVxx.Complexity='real';
      | structVxx.SamplingMode='Sample based';
      | structVxx.SampleTime=-1;
      | assignin('base',DataName,structVxx);
      settings: AttributesFormatString=%<MaskType>  RTWSystemCode=Nonreusable function  RTWFcnNameOpts=User specified
      mask Help:
      | eval('path_lib=fileparts(which(''AEMS_Standard_Library''));');
      | mskblk=get_param(gcbh,'MaskType');
      | doc_path = [path_lib '\Help\',mskblk,'.pdf'];
      | eval('open(doc_path)');
  AEMS_SUPPLIER_CALL_TI_MINI_OK_LPOS : Subsystem  Tag=[LIB]  TreatAsAtomicUnit=on  RTWFcnName=SUPPLIER_CALL_Ti_mini_ok_lpos  mask(AEMS_SUPPLIER_CALL_TI_MINI_OK_LPOS){}
      mask help:
      | Verify if the estimated fuel injection ti is over minimum possible ti.
      |
      | This block is to call Supplier call API.
      mask init:
      | Thisblk = gcb;
      | model_type_pos = strsplit(Thisblk,'/');%to split all the layer paths in order to get the runnable path
      | runnable_path = [bdroot '/' model_type_pos{2}];%to get the runnable or AIPCALL path
      | trg_port_name = get_param(find_system(runnable_path,'BlockType','TriggerPort'),'Name');%to get the function call trigger name
      | TaskRate = '';%the raster suffix is stored in the parameter 
      | 
      | if ~isempty(trg_port_name)
      |     trg_port_name_spltd = strsplit(trg_port_name{1},'_');%splitting is done in order to get the raster and its type(Sched or Event)
      |     
      |     % checking for rasters of type Sched or Event especially occuring in
      |     % runnables
      |     if ~isempty(regexp(trg_port_name_spltd{1},'^Sched|^Event','once')) 
      |         TaskRate = ['_' regexprep(trg_port_name_spltd{1},'Sched|Event','','once')];
      |         
      |     %checking if the raster is dcmcb and this is applicable only for
      |     %APICALL
      |     elseif ~isempty(regexp([trg_port_name_spltd{1} '_' trg_port_name_spltd{2} '_' ],'^DataServices_DCM_|^RoutineServices_DCM_','once'))||...
      |             ~isempty(regexp(trg_port_name_spltd{1},'^Dcm$','once'))
      |         TaskRate = '_dcmcb';
      |         
      |     %checking if this block is used under the function call trigger
      |     %starting with "Com" and then giving an error message
      |     %this is applicable only for APICALL
      |     elseif ~isempty(regexp(trg_port_name_spltd{1},'^Com$','once'))
      |         msg = sprintf(['\n','The Supplier call block "' Thisblk '" should not be present within APICALLs having function call trigger as "Com"']);
      |         errordlg(msg);
      |         return;
      |     end
      | end
      | 
      | DataName = ['Supplier_call_ti_mini_ok_lpos' TaskRate];%the variable name that should be given to DataStoreRead block 
      | set_param([Thisblk '/Data Store Read'],'DataStoreName',DataName);%Setting the DataStoreName of DataStoreRead block
      | 
      | %other settings done to this variable name
      | structVxx=Simulink.Signal;
      | structVxx.Dimensions=1;
      | structVxx.DimensionsMode='Fixed';
      | structVxx.DataType='boolean';
      | structVxx.Complexity='real';
      | structVxx.SamplingMode='Sample based';
      | structVxx.SampleTime=-1;
      | assignin('base',DataName,structVxx);
      settings: AttributesFormatString=%<MaskType>  RTWSystemCode=Nonreusable function  RTWFcnNameOpts=User specified
      mask Help:
      | eval('path_lib=fileparts(which(''AEMS_Standard_Library''));');
      | mskblk=get_param(gcbh,'MaskType');
      | doc_path = [path_lib '\Help\',mskblk,'.pdf'];
      | eval('open(doc_path)');
  AEMS_SUPPLIER_CALL_TI_MINI_OK_LPOS1_2SL : Subsystem  Tag=[LIB]  TreatAsAtomicUnit=on  RTWFcnName=SUPPLIER_CALL_Ti_mini_ok_lpos1_2sl  mask(AEMS_SUPPLIER_CALL_TI_MINI_OK_LPOS1_2SL){}
      mask help:
      | Verify if the estimated fuel injection ti is over minimum possible ti.
      |
      | This block is to call Supplier call API.
      mask init:
      | Thisblk = gcb;
      | model_type_pos = strsplit(Thisblk,'/');%to split all the layer paths in order to get the runnable path
      | runnable_path = [bdroot '/' model_type_pos{2}];%to get the runnable or AIPCALL path
      | trg_port_name = get_param(find_system(runnable_path,'BlockType','TriggerPort'),'Name');%to get the function call trigger name
      | TaskRate = '';%the raster suffix is stored in the parameter 
      | 
      | if ~isempty(trg_port_name)
      |     trg_port_name_spltd = strsplit(trg_port_name{1},'_');%splitting is done in order to get the raster and its type(Sched or Event)
      |     
      |     % checking for rasters of type Sched or Event especially occuring in
      |     % runnables
      |     if ~isempty(regexp(trg_port_name_spltd{1},'^Sched|^Event','once')) 
      |         TaskRate = ['_' regexprep(trg_port_name_spltd{1},'Sched|Event','','once')];
      |         
      |     %checking if the raster is dcmcb and this is applicable only for
      |     %APICALL
      |     elseif ~isempty(regexp([trg_port_name_spltd{1} '_' trg_port_name_spltd{2} '_' ],'^DataServices_DCM_|^RoutineServices_DCM_','once'))||...
      |             ~isempty(regexp(trg_port_name_spltd{1},'^Dcm$','once'))
      |         TaskRate = '_dcmcb';
      |         
      |     %checking if this block is used under the function call trigger
      |     %starting with "Com" and then giving an error message
      |     %this is applicable only for APICALL
      |     elseif ~isempty(regexp(trg_port_name_spltd{1},'^Com$','once'))
      |         msg = sprintf(['\n','The Supplier call block "' Thisblk '" should not be present within APICALLs having function call trigger as "Com"']);
      |         errordlg(msg);
      |         return;
      |     end
      | end
      | 
      | DataName = ['Supplier_call_ti_mini_ok_lpos1' TaskRate];%the variable name that should be given to DataStoreRead block 
      | set_param([Thisblk '/Data Store Read'],'DataStoreName',DataName);%Setting the DataStoreName of DataStoreRead block
      | 
      | %other settings done to this variable name
      | structVxx=Simulink.Signal;
      | structVxx.Dimensions=1;
      | structVxx.DimensionsMode='Fixed';
      | structVxx.DataType='boolean';
      | structVxx.Complexity='real';
      | structVxx.SamplingMode='Sample based';
      | structVxx.SampleTime=-1;
      | assignin('base',DataName,structVxx);
      settings: AttributesFormatString=%<MaskType>  RTWSystemCode=Nonreusable function  RTWFcnNameOpts=User specified
      mask Help:
      | eval('path_lib=fileparts(which(''AEMS_Standard_Library''));');
      | mskblk=get_param(gcbh,'MaskType');
      | doc_path = [path_lib '\Help\',mskblk,'.pdf'];
      | eval('open(doc_path)');
  AEMS_SUPPLIER_CALL_TI_MINI_OK_LPOS1_3SL : Subsystem  Tag=[LIB]  TreatAsAtomicUnit=on  RTWFcnName=SUPPLIER_CALL_Ti_mini_ok_lpos1_3sl  mask(AEMS_SUPPLIER_CALL_TI_MINI_OK_LPOS1_3SL){}
      mask help:
      | Verify if the estimated fuel injection ti is over minimum possible ti.
      |
      | This block is to call Supplier call API.
      mask init: same as AEMS_Standard_Library/SPECIFIC/AEMS_SUPPLIER_CALL_TI_MINI_OK_LPOS1_2SL
      settings: AttributesFormatString=%<MaskType>  RTWSystemCode=Nonreusable function  RTWFcnNameOpts=User specified
      mask Help:
      | eval('path_lib=fileparts(which(''AEMS_Standard_Library''));');
      | mskblk=get_param(gcbh,'MaskType');
      | doc_path = [path_lib '\Help\',mskblk,'.pdf'];
      | eval('open(doc_path)');
  AEMS_SUPPLIER_CALL_TI_MINI_OK_LPOS1_4SL : Subsystem  Tag=[LIB]  TreatAsAtomicUnit=on  RTWFcnName=SUPPLIER_CALL_Ti_mini_ok_lpos1_4sl  mask(AEMS_SUPPLIER_CALL_TI_MINI_OK_LPOS1_4SL){}
      mask help:
      | Verify if the estimated fuel injection ti is over minimum possible ti.
      |
      | This block is to call Supplier call API.
      mask init:
      | Thisblk = gcb;
      | model_type_pos = strsplit(Thisblk,'/');%to split all the layer paths in order to get the runnable path
      | runnable_path = [bdroot '/' model_type_pos{2}];%to get the runnable or AIPCALL path
      | trg_port_name = get_param(find_system(runnable_path,'BlockType','TriggerPort'),'Name');%to get the function call trigger name
      | TaskRate = '';%the raster suffix is stored in the parameter 
      | 
      | if ~isempty(trg_port_name)
      |     trg_port_name_spltd = strsplit(trg_port_name{1},'_');%splitting is done in order to get the raster and its type(Sched or Event)
      |     
      |     % checking for rasters of type Sched or Event especially occuring in
      |     % runnables
      |     if ~isempty(regexp(trg_port_name_spltd{1},'^Sched|^Event','once')) 
      |         TaskRate = ['_' regexprep(trg_port_name_spltd{1},'Sched|Event','','once')];
      |         
      |     %checking if the raster is dcmcb and this is applicable only for
      |     %APICALL
      |     elseif ~isempty(regexp([trg_port_name_spltd{1} '_' trg_port_name_spltd{2} '_' ],'^DataServices_DCM_|^RoutineServices_DCM_','once'))||...
      |             ~isempty(regexp(trg_port_name_spltd{1},'^Dcm$','once'))
      |         TaskRate = '_dcmcb';
      |         
      |     %checking if this block is used under the function call trigger
      |     %starting with "Com" and then giving an error message
      |     %this is applicable only for APICALL
      |     elseif ~isempty(regexp(trg_port_name_spltd{1},'^Com$','once'))
      |         msg = sprintf(['\n','The Supplier call block "' Thisblk '" should not be present within APICALLs having function call trigger as "Com"']);
      |         errordlg(msg);
      |         return;
      |     end
      | end
      | 
      | DataName = ['Supplier_call_ti_mini_ok_lpos1' TaskRate];%the variable name that should be given to DataStoreRead block 
      | set_param([Thisblk '/Data Store Read'],'DataStoreName',DataName);%Setting the DataStoreName of DataStoreRead block
      | 
      | %other settings done to this variable name
      | structVxx=Simulink.Signal;
      | structVxx.Dimensions=1;
      | structVxx.DimensionsMode='Fixed';
      | structVxx.DataType='boolean';
      | structVxx.Complexity='real';
      | structVxx.SamplingMode='Sample based';
      | structVxx.SampleTime=-1;
      | assignin('base',DataName,structVxx);
      settings: AttributesFormatString=%<MaskType>  RTWSystemCode=Nonreusable function  RTWFcnNameOpts=User specified
      mask Help:
      | eval('path_lib=fileparts(which(''AEMS_Standard_Library''));');
      | mskblk=get_param(gcbh,'MaskType');
      | doc_path = [path_lib '\Help\',mskblk,'.pdf'];
      | eval('open(doc_path)');
  AEMS_SUPPLIER_CALL_TI_MINI_OK_LPOS2_2SL : Subsystem  Tag=[LIB]  TreatAsAtomicUnit=on  RTWFcnName=SUPPLIER_CALL_Ti_mini_ok_lpos2_2sl  mask(AEMS_SUPPLIER_CALL_TI_MINI_OK_LPOS2_2SL){}
      mask help:
      | Verify if the estimated fuel injection ti is over minimum possible ti.
      |
      | This block is to call Supplier call API.
      mask init:
      | Thisblk = gcb;
      | model_type_pos = strsplit(Thisblk,'/');%to split all the layer paths in order to get the runnable path
      | runnable_path = [bdroot '/' model_type_pos{2}];%to get the runnable or AIPCALL path
      | trg_port_name = get_param(find_system(runnable_path,'BlockType','TriggerPort'),'Name');%to get the function call trigger name
      | TaskRate = '';%the raster suffix is stored in the parameter 
      | 
      | if ~isempty(trg_port_name)
      |     trg_port_name_spltd = strsplit(trg_port_name{1},'_');%splitting is done in order to get the raster and its type(Sched or Event)
      |     
      |     % checking for rasters of type Sched or Event especially occuring in
      |     % runnables
      |     if ~isempty(regexp(trg_port_name_spltd{1},'^Sched|^Event','once')) 
      |         TaskRate = ['_' regexprep(trg_port_name_spltd{1},'Sched|Event','','once')];
      |         
      |     %checking if the raster is dcmcb and this is applicable only for
      |     %APICALL
      |     elseif ~isempty(regexp([trg_port_name_spltd{1} '_' trg_port_name_spltd{2} '_' ],'^DataServices_DCM_|^RoutineServices_DCM_','once'))||...
      |             ~isempty(regexp(trg_port_name_spltd{1},'^Dcm$','once'))
      |         TaskRate = '_dcmcb';
      |         
      |     %checking if this block is used under the function call trigger
      |     %starting with "Com" and then giving an error message
      |     %this is applicable only for APICALL
      |     elseif ~isempty(regexp(trg_port_name_spltd{1},'^Com$','once'))
      |         msg = sprintf(['\n','The Supplier call block "' Thisblk '" should not be present within APICALLs having function call trigger as "Com"']);
      |         errordlg(msg);
      |         return;
      |     end
      | end
      | 
      | DataName = ['Supplier_call_ti_mini_ok_lpos2' TaskRate];%the variable name that should be given to DataStoreRead block 
      | set_param([Thisblk '/Data Store Read'],'DataStoreName',DataName);%Setting the DataStoreName of DataStoreRead block
      | 
      | %other settings done to this variable name
      | structVxx=Simulink.Signal;
      | % structVxx=Simulink.Signal;
      | structVxx.Dimensions=1;
      | structVxx.DimensionsMode='Fixed';
      | structVxx.DataType='boolean';
      | structVxx.Complexity='real';
      | structVxx.SamplingMode='Sample based';
      | structVxx.SampleTime=-1;
      | assignin('base',DataName,structVxx);
      settings: AttributesFormatString=%<MaskType>  RTWSystemCode=Nonreusable function  RTWFcnNameOpts=User specified
      mask Help:
      | eval('path_lib=fileparts(which(''AEMS_Standard_Library''));');
      | mskblk=get_param(gcbh,'MaskType');
      | doc_path = [path_lib '\Help\',mskblk,'.pdf'];
      | eval('open(doc_path)');
  AEMS_SUPPLIER_CALL_TI_MINI_OK_LPOS2_3SL : Subsystem  Tag=[LIB]  TreatAsAtomicUnit=on  RTWFcnName=SUPPLIER_CALL_Ti_mini_ok_lpos2_3sl  mask(AEMS_SUPPLIER_CALL_TI_MINI_OK_LPOS2_3SL){}
      mask help:
      | Verify if the estimated fuel injection ti is over minimum possible ti.
      |
      | This block is to call Supplier call API.
      mask init:
      | Thisblk = gcb;
      | model_type_pos = strsplit(Thisblk,'/');%to split all the layer paths in order to get the runnable path
      | runnable_path = [bdroot '/' model_type_pos{2}];%to get the runnable or AIPCALL path
      | trg_port_name = get_param(find_system(runnable_path,'BlockType','TriggerPort'),'Name');%to get the function call trigger name
      | TaskRate = '';%the raster suffix is stored in the parameter 
      | 
      | if ~isempty(trg_port_name)
      |     trg_port_name_spltd = strsplit(trg_port_name{1},'_');%splitting is done in order to get the raster and its type(Sched or Event)
      |     
      |     % checking for rasters of type Sched or Event especially occuring in
      |     % runnables
      |     if ~isempty(regexp(trg_port_name_spltd{1},'^Sched|^Event','once')) 
      |         TaskRate = ['_' regexprep(trg_port_name_spltd{1},'Sched|Event','','once')];
      |         
      |     %checking if the raster is dcmcb and this is applicable only for
      |     %APICALL
      |     elseif ~isempty(regexp([trg_port_name_spltd{1} '_' trg_port_name_spltd{2} '_' ],'^DataServices_DCM_|^RoutineServices_DCM_','once'))||...
      |             ~isempty(regexp(trg_port_name_spltd{1},'^Dcm$','once'))
      |         TaskRate = '_dcmcb';
      |         
      |     %checking if this block is used under the function call trigger
      |     %starting with "Com" and then giving an error message
      |     %this is applicable only for APICALL
      |     elseif ~isempty(regexp(trg_port_name_spltd{1},'^Com$','once'))
      |         msg = sprintf(['\n','The Supplier call block "' Thisblk '" should not be present within APICALLs having function call trigger as "Com"']);
      |         errordlg(msg);
      |         return;
      |     end
      | end
      | 
      | DataName = ['Supplier_call_ti_mini_ok_lpos2' TaskRate];%the variable name that should be given to DataStoreRead block 
      | set_param([Thisblk '/Data Store Read'],'DataStoreName',DataName);%Setting the DataStoreName of DataStoreRead block
      | 
      | %other settings done to this variable name
      | structVxx=Simulink.Signal;
      | structVxx.Dimensions=1;
      | structVxx.DimensionsMode='Fixed';
      | structVxx.DataType='boolean';
      | structVxx.Complexity='real';
      | structVxx.SamplingMode='Sample based';
      | structVxx.SampleTime=-1;
      | assignin('base',DataName,structVxx);
      settings: AttributesFormatString=%<MaskType>  RTWSystemCode=Nonreusable function  RTWFcnNameOpts=User specified
      mask Help:
      | eval('path_lib=fileparts(which(''AEMS_Standard_Library''));');
      | mskblk=get_param(gcbh,'MaskType');
      | doc_path = [path_lib '\Help\',mskblk,'.pdf'];
      | eval('open(doc_path)');
  AEMS_SUPPLIER_CALL_TI_MINI_OK_LPOS2_4SL : Subsystem  Tag=[LIB]  TreatAsAtomicUnit=on  RTWFcnName=SUPPLIER_CALL_Ti_mini_ok_lpos2_4sl  mask(AEMS_SUPPLIER_CALL_TI_MINI_OK_LPOS2_4SL){}
      mask help:
      | Verify if the estimated fuel injection ti is over minimum possible ti.
      |
      | This block is to call Supplier call API.
      mask init:
      | Thisblk = gcb;
      | model_type_pos = strsplit(Thisblk,'/');%to split all the layer paths in order to get the runnable path
      | runnable_path = [bdroot '/' model_type_pos{2}];%to get the runnable or AIPCALL path
      | trg_port_name = get_param(find_system(runnable_path,'BlockType','TriggerPort'),'Name');%to get the function call trigger name
      | TaskRate = '';%the raster suffix is stored in the parameter 
      | 
      | if ~isempty(trg_port_name)
      |     trg_port_name_spltd = strsplit(trg_port_name{1},'_');%splitting is done in order to get the raster and its type(Sched or Event)
      |     
      |     % checking for rasters of type Sched or Event especially occuring in
      |     % runnables
      |     if ~isempty(regexp(trg_port_name_spltd{1},'^Sched|^Event','once')) 
      |         TaskRate = ['_' regexprep(trg_port_name_spltd{1},'Sched|Event','','once')];
      |         
      |     %checking if the raster is dcmcb and this is applicable only for
      |     %APICALL
      |     elseif ~isempty(regexp([trg_port_name_spltd{1} '_' trg_port_name_spltd{2} '_' ],'^DataServices_DCM_|^RoutineServices_DCM_','once'))||...
      |             ~isempty(regexp(trg_port_name_spltd{1},'^Dcm$','once'))
      |         TaskRate = '_dcmcb';
      |         
      |     %checking if this block is used under the function call trigger
      |     %starting with "Com" and then giving an error message
      |     %this is applicable only for APICALL
      |     elseif ~isempty(regexp(trg_port_name_spltd{1},'^Com$','once'))
      |         msg = sprintf(['\n','The Supplier call block "' Thisblk '" should not be present within APICALLs having function call trigger as "Com"']);
      |         errordlg(msg);
      |         return;
      |     end
      | end
      | 
      | DataName = ['Supplier_call_ti_mini_ok_lpos3' TaskRate];%the variable name that should be given to DataStoreRead block 
      | set_param([Thisblk '/Data Store Read'],'DataStoreName',DataName);%Setting the DataStoreName of DataStoreRead block
      | 
      | %other settings done to this variable name
      | structVxx=Simulink.Signal;
      | structVxx.Dimensions=1;
      | structVxx.DimensionsMode='Fixed';
      | structVxx.DataType='boolean';
      | structVxx.Complexity='real';
      | structVxx.SamplingMode='Sample based';
      | structVxx.SampleTime=-1;
      | assignin('base',DataName,structVxx);
      settings: AttributesFormatString=%<MaskType>  RTWSystemCode=Nonreusable function  RTWFcnNameOpts=User specified
      mask Help:
      | eval('path_lib=fileparts(which(''AEMS_Standard_Library''));');
      | mskblk=get_param(gcbh,'MaskType');
      | doc_path = [path_lib '\Help\',mskblk,'.pdf'];
      | eval('open(doc_path)');
  AEMS_SUPPLIER_CALL_TI_MINI_OK_LPOS3_3SL : Subsystem  Tag=[LIB]  TreatAsAtomicUnit=on  RTWFcnName=SUPPLIER_CALL_Ti_mini_ok_lpos3_3sl  mask(AEMS_SUPPLIER_CALL_TI_MINI_OK_LPOS3_3SL){}
      mask help:
      | Verify if the estimated fuel injection ti is over minimum possible ti.
      |
      | This block is to call Supplier call API.
      mask init: same as AEMS_Standard_Library/SPECIFIC/AEMS_SUPPLIER_CALL_TI_MINI_OK_LPOS2_4SL
      settings: AttributesFormatString=%<MaskType>  RTWSystemCode=Nonreusable function  RTWFcnNameOpts=User specified
      mask Help:
      | eval('path_lib=fileparts(which(''AEMS_Standard_Library''));');
      | mskblk=get_param(gcbh,'MaskType');
      | doc_path = [path_lib '\Help\',mskblk,'.pdf'];
      | eval('open(doc_path)');
  AEMS_SUPPLIER_CALL_TI_MINI_OK_LPOS3_4SL : Subsystem  Tag=[LIB]  TreatAsAtomicUnit=on  RTWFcnName=SUPPLIER_CALL_Ti_mini_ok_lpos3_4sl  mask(AEMS_SUPPLIER_CALL_TI_MINI_OK_LPOS3_4SL){}
      mask help:
      | Verify if the estimated fuel injection ti is over minimum possible ti.
      |
      | This block is to call Supplier call API.
      mask init:
      | Thisblk = gcb;
      | model_type_pos = strsplit(Thisblk,'/');%to split all the layer paths in order to get the runnable path
      | runnable_path = [bdroot '/' model_type_pos{2}];%to get the runnable or AIPCALL path
      | trg_port_name = get_param(find_system(runnable_path,'BlockType','TriggerPort'),'Name');%to get the function call trigger name
      | TaskRate = '';%the raster suffix is stored in the parameter 
      | 
      | if ~isempty(trg_port_name)
      |     trg_port_name_spltd = strsplit(trg_port_name{1},'_');%splitting is done in order to get the raster and its type(Sched or Event)
      |     
      |     % checking for rasters of type Sched or Event especially occuring in
      |     % runnables
      |     if ~isempty(regexp(trg_port_name_spltd{1},'^Sched|^Event','once')) 
      |         TaskRate = ['_' regexprep(trg_port_name_spltd{1},'Sched|Event','','once')];
      |         
      |     %checking if the raster is dcmcb and this is applicable only for
      |     %APICALL
      |     elseif ~isempty(regexp([trg_port_name_spltd{1} '_' trg_port_name_spltd{2} '_' ],'^DataServices_DCM_|^RoutineServices_DCM_','once'))||...
      |             ~isempty(regexp(trg_port_name_spltd{1},'^Dcm$','once'))
      |         TaskRate = '_dcmcb';
      |         
      |     %checking if this block is used under the function call trigger
      |     %starting with "Com" and then giving an error message
      |     %this is applicable only for APICALL
      |     elseif ~isempty(regexp(trg_port_name_spltd{1},'^Com$','once'))
      |         msg = sprintf(['\n','The Supplier call block "' Thisblk '" should not be present within APICALLs having function call trigger as "Com"']);
      |         errordlg(msg);
      |         return;
      |     end
      | end
      | 
      | DataName = ['Supplier_call_ti_mini_ok_lpos2' TaskRate];%the variable name that should be given to DataStoreRead block 
      | set_param([Thisblk '/Data Store Read'],'DataStoreName',DataName);%Setting the DataStoreName of DataStoreRead block
      | 
      | %other settings done to this variable name
      | structVxx=Simulink.Signal;
      | structVxx.Dimensions=1;
      | structVxx.DimensionsMode='Fixed';
      | structVxx.DataType='boolean';
      | structVxx.Complexity='real';
      | structVxx.SamplingMode='Sample based';
      | structVxx.SampleTime=-1;
      | assignin('base',DataName,structVxx);
      settings: AttributesFormatString=%<MaskType>  RTWSystemCode=Nonreusable function  RTWFcnNameOpts=User specified
      mask Help:
      | eval('path_lib=fileparts(which(''AEMS_Standard_Library''));');
      | mskblk=get_param(gcbh,'MaskType');
      | doc_path = [path_lib '\Help\',mskblk,'.pdf'];
      | eval('open(doc_path)');
  AEMS_SUPPLIER_CALL_TI_MINI_OK_LPOS4_4SL : Subsystem  Tag=[LIB]  TreatAsAtomicUnit=on  RTWFcnName=SUPPLIER_CALL_Ti_mini_ok_lpos4_4sl  mask(AEMS_SUPPLIER_CALL_TI_MINI_OK_LPOS4_4SL){}
      mask help:
      | Verify if the estimated fuel injection ti is over minimum possible ti.
      |
      | This block is to call Supplier call API.
      mask init:
      | Thisblk = gcb;
      | model_type_pos = strsplit(Thisblk,'/');%to split all the layer paths in order to get the runnable path
      | runnable_path = [bdroot '/' model_type_pos{2}];%to get the runnable or AIPCALL path
      | trg_port_name = get_param(find_system(runnable_path,'BlockType','TriggerPort'),'Name');%to get the function call trigger name
      | TaskRate = '';%the raster suffix is stored in the parameter 
      | 
      | if ~isempty(trg_port_name)
      |     trg_port_name_spltd = strsplit(trg_port_name{1},'_');%splitting is done in order to get the raster and its type(Sched or Event)
      |     
      |     % checking for rasters of type Sched or Event especially occuring in
      |     % runnables
      |     if ~isempty(regexp(trg_port_name_spltd{1},'^Sched|^Event','once')) 
      |         TaskRate = ['_' regexprep(trg_port_name_spltd{1},'Sched|Event','','once')];
      |         
      |     %checking if the raster is dcmcb and this is applicable only for
      |     %APICALL
      |     elseif ~isempty(regexp([trg_port_name_spltd{1} '_' trg_port_name_spltd{2} '_' ],'^DataServices_DCM_|^RoutineServices_DCM_','once'))||...
      |             ~isempty(regexp(trg_port_name_spltd{1},'^Dcm$','once'))
      |         TaskRate = '_dcmcb';
      |         
      |     %checking if this block is used under the function call trigger
      |     %starting with "Com" and then giving an error message
      |     %this is applicable only for APICALL
      |     elseif ~isempty(regexp(trg_port_name_spltd{1},'^Com$','once'))
      |         msg = sprintf(['\n','The Supplier call block "' Thisblk '" should not be present within APICALLs having function call trigger as "Com"']);
      |         errordlg(msg);
      |         return;
      |     end
      | end
      | 
      | DataName = ['Supplier_call_ti_mini_ok_lpos4' TaskRate];%the variable name that should be given to DataStoreRead block 
      | set_param([Thisblk '/Data Store Read'],'DataStoreName',DataName);%Setting the DataStoreName of DataStoreRead block
      | 
      | %other settings done to this variable name
      | structVxx=Simulink.Signal;
      | structVxx.Dimensions=1;
      | structVxx.DimensionsMode='Fixed';
      | structVxx.DataType='boolean';
      | structVxx.Complexity='real';
      | structVxx.SamplingMode='Sample based';
      | structVxx.SampleTime=-1;
      | assignin('base',DataName,structVxx);
      settings: AttributesFormatString=%<MaskType>  RTWSystemCode=Nonreusable function  RTWFcnNameOpts=User specified
      mask Help:
      | eval('path_lib=fileparts(which(''AEMS_Standard_Library''));');
      | mskblk=get_param(gcbh,'MaskType');
      | doc_path = [path_lib '\Help\',mskblk,'.pdf'];
      | eval('open(doc_path)');
  AEMS_SUPPLIER_CALL_TI_MINI_OK_MAIN : Subsystem  Tag=[LIB]  TreatAsAtomicUnit=on  RTWFcnName=SUPPLIER_CALL_Ti_mini_ok_main  mask(AEMS_SUPPLIER_CALL_TI_MINI_OK_MAIN){}
      mask help:
      | Verify if the estimated fuel injection ti is over minimum possible ti.
      |
      | This block is to call Supplier call API.
      mask init:
      | Thisblk = gcb;
      | model_type_pos = strsplit(Thisblk,'/');%to split all the layer paths in order to get the runnable path
      | runnable_path = [bdroot '/' model_type_pos{2}];%to get the runnable or AIPCALL path
      | trg_port_name = get_param(find_system(runnable_path,'BlockType','TriggerPort'),'Name');%to get the function call trigger name
      | TaskRate = '';%the raster suffix is stored in the parameter 
      | 
      | if ~isempty(trg_port_name)
      |     trg_port_name_spltd = strsplit(trg_port_name{1},'_');%splitting is done in order to get the raster and its type(Sched or Event)
      |     
      |     % checking for rasters of type Sched or Event especially occuring in
      |     % runnables
      |     if ~isempty(regexp(trg_port_name_spltd{1},'^Sched|^Event','once')) 
      |         TaskRate = ['_' regexprep(trg_port_name_spltd{1},'Sched|Event','','once')];
      |         
      |     %checking if the raster is dcmcb and this is applicable only for
      |     %APICALL
      |     elseif ~isempty(regexp([trg_port_name_spltd{1} '_' trg_port_name_spltd{2} '_' ],'^DataServices_DCM_|^RoutineServices_DCM_','once'))||...
      |             ~isempty(regexp(trg_port_name_spltd{1},'^Dcm$','once'))
      |         TaskRate = '_dcmcb';
      |         
      |     %checking if this block is used under the function call trigger
      |     %starting with "Com" and then giving an error message
      |     %this is applicable only for APICALL
      |     elseif ~isempty(regexp(trg_port_name_spltd{1},'^Com$','once'))
      |         msg = sprintf(['\n','The Supplier call block "' Thisblk '" should not be present within APICALLs having function call trigger as "Com"']);
      |         errordlg(msg);
      |         return;
      |     end
      | end
      | 
      | DataName = ['Supplier_call_ti_mini_ok_main' TaskRate];%the variable name that should be given to DataStoreRead block 
      | set_param([Thisblk '/Data Store Read'],'DataStoreName',DataName);%Setting the DataStoreName of DataStoreRead block
      | 
      | %other settings done to this variable name
      | structVxx=Simulink.Signal;
      | structVxx.Dimensions=1;
      | structVxx.DimensionsMode='Fixed';
      | structVxx.DataType='boolean';
      | structVxx.Complexity='real';
      | structVxx.SamplingMode='Sample based';
      | structVxx.SampleTime=-1;
      | assignin('base',DataName,structVxx);
      settings: AttributesFormatString=%<MaskType>  RTWSystemCode=Nonreusable function  RTWFcnNameOpts=User specified
      mask Help:
      | eval('path_lib=fileparts(which(''AEMS_Standard_Library''));');
      | mskblk=get_param(gcbh,'MaskType');
      | doc_path = [path_lib '\Help\',mskblk,'.pdf'];
      | eval('open(doc_path)');
  AEMS_SUPPLIER_CALL_TI_MINI_OK_PINJ1 : Subsystem  Tag=[LIB]  TreatAsAtomicUnit=on  RTWFcnName=SUPPLIER_CALL_Ti_mini_ok_pinj1  mask(AEMS_SUPPLIER_CALL_TI_MINI_OK_PINJ1){}
      mask help:
      | Verify if the estimated fuel injection ti is over minimum possible ti.
      |
      | This block is to call Supplier call API.
      mask init:
      | Thisblk = gcb;
      | model_type_pos = strsplit(Thisblk,'/');%to split all the layer paths in order to get the runnable path
      | runnable_path = [bdroot '/' model_type_pos{2}];%to get the runnable or AIPCALL path
      | trg_port_name = get_param(find_system(runnable_path,'BlockType','TriggerPort'),'Name');%to get the function call trigger name
      | TaskRate = '';%the raster suffix is stored in the parameter 
      | 
      | if ~isempty(trg_port_name)
      |     trg_port_name_spltd = strsplit(trg_port_name{1},'_');%splitting is done in order to get the raster and its type(Sched or Event)
      |     
      |     % checking for rasters of type Sched or Event especially occuring in
      |     % runnables
      |     if ~isempty(regexp(trg_port_name_spltd{1},'^Sched|^Event','once')) 
      |         TaskRate = ['_' regexprep(trg_port_name_spltd{1},'Sched|Event','','once')];
      |         
      |     %checking if the raster is dcmcb and this is applicable only for
      |     %APICALL
      |     elseif ~isempty(regexp([trg_port_name_spltd{1} '_' trg_port_name_spltd{2} '_' ],'^DataServices_DCM_|^RoutineServices_DCM_','once'))||...
      |             ~isempty(regexp(trg_port_name_spltd{1},'^Dcm$','once'))
      |         TaskRate = '_dcmcb';
      |         
      |     %checking if this block is used under the function call trigger
      |     %starting with "Com" and then giving an error message
      |     %this is applicable only for APICALL
      |     elseif ~isempty(regexp(trg_port_name_spltd{1},'^Com$','once'))
      |         msg = sprintf(['\n','The Supplier call block "' Thisblk '" should not be present within APICALLs having function call trigger as "Com"']);
      |         errordlg(msg);
      |         return;
      |     end
      | end
      | 
      | DataName = ['Supplier_call_ti_mini_ok_pinj1' TaskRate];%the variable name that should be given to DataStoreRead block 
      | set_param([Thisblk '/Data Store Read'],'DataStoreName',DataName);%Setting the DataStoreName of DataStoreRead block
      | 
      | %other settings done to this variable name
      | structVxx=Simulink.Signal;
      | structVxx.Dimensions=1;
      | structVxx.DimensionsMode='Fixed';
      | structVxx.DataType='boolean';
      | structVxx.Complexity='real';
      | structVxx.SamplingMode='Sample based';
      | structVxx.SampleTime=-1;
      | assignin('base',DataName,structVxx);
      settings: AttributesFormatString=%<MaskType>  RTWSystemCode=Nonreusable function  RTWFcnNameOpts=User specified
      mask Help:
      | eval('path_lib=fileparts(which(''AEMS_Standard_Library''));');
      | mskblk=get_param(gcbh,'MaskType');
      | doc_path = [path_lib '\Help\',mskblk,'.pdf'];
      | eval('open(doc_path)');
  AEMS_SUPPLIER_CALL_TI_MINI_OK_PINJ2 : Subsystem  Tag=[LIB]  TreatAsAtomicUnit=on  RTWFcnName=SUPPLIER_CALL_Ti_mini_ok_pinj2  mask(AEMS_SUPPLIER_CALL_TI_MINI_OK_PINJ2){}
      mask help:
      | Verify if the estimated fuel injection ti is over minimum possible ti.
      |
      | This block is to call Supplier call API
      mask init:
      | Thisblk = gcb;
      | model_type_pos = strsplit(Thisblk,'/');%to split all the layer paths in order to get the runnable path
      | runnable_path = [bdroot '/' model_type_pos{2}];%to get the runnable or AIPCALL path
      | trg_port_name = get_param(find_system(runnable_path,'BlockType','TriggerPort'),'Name');%to get the function call trigger name
      | TaskRate = '';%the raster suffix is stored in the parameter 
      | 
      | if ~isempty(trg_port_name)
      |     trg_port_name_spltd = strsplit(trg_port_name{1},'_');%splitting is done in order to get the raster and its type(Sched or Event)
      |     
      |     % checking for rasters of type Sched or Event especially occuring in
      |     % runnables
      |     if ~isempty(regexp(trg_port_name_spltd{1},'^Sched|^Event','once')) 
      |         TaskRate = ['_' regexprep(trg_port_name_spltd{1},'Sched|Event','','once')];
      |         
      |     %checking if the raster is dcmcb and this is applicable only for
      |     %APICALL
      |     elseif ~isempty(regexp([trg_port_name_spltd{1} '_' trg_port_name_spltd{2} '_' ],'^DataServices_DCM_|^RoutineServices_DCM_','once'))||...
      |             ~isempty(regexp(trg_port_name_spltd{1},'^Dcm$','once'))
      |         TaskRate = '_dcmcb';
      |         
      |     %checking if this block is used under the function call trigger
      |     %starting with "Com" and then giving an error message
      |     %this is applicable only for APICALL
      |     elseif ~isempty(regexp(trg_port_name_spltd{1},'^Com$','once'))
      |         msg = sprintf(['\n','The Supplier call block "' Thisblk '" should not be present within APICALLs having function call trigger as "Com"']);
      |         errordlg(msg);
      |         return;
      |     end
      | end
      | 
      | DataName = ['Supplier_call_ti_mini_ok_pinj2' TaskRate];%the variable name that should be given to DataStoreRead block 
      | set_param([Thisblk '/Data Store Read'],'DataStoreName',DataName);%Setting the DataStoreName of DataStoreRead block
      | 
      | %other settings done to this variable name
      | structVxx=Simulink.Signal;
      | structVxx.Dimensions=1;
      | structVxx.DimensionsMode='Fixed';
      | structVxx.DataType='boolean';
      | structVxx.Complexity='real';
      | structVxx.SamplingMode='Sample based';
      | structVxx.SampleTime=-1;
      | assignin('base',DataName,structVxx);
      settings: AttributesFormatString=%<MaskType>  RTWSystemCode=Nonreusable function  RTWFcnNameOpts=User specified
      mask Help:
      | eval('path_lib=fileparts(which(''AEMS_Standard_Library''));');
      | mskblk=get_param(gcbh,'MaskType');
      | doc_path = [path_lib '\Help\',mskblk,'.pdf'];
      | eval('open(doc_path)');
  AEMS_SUPPLIER_CALL_TI_MINI_OK_PINJ3 : Subsystem  Tag=[LIB]  TreatAsAtomicUnit=on  RTWFcnName=SUPPLIER_CALL_Ti_mini_ok_pinj3  mask(AEMS_SUPPLIER_CALL_TI_MINI_OK_PINJ3){}
      mask help:
      | Verify if the estimated fuel injection ti is over minimum possible ti.
      |
      | This block is to call Supplier call API.
      mask init:
      | Thisblk = gcb;
      | model_type_pos = strsplit(Thisblk,'/');%to split all the layer paths in order to get the runnable path
      | runnable_path = [bdroot '/' model_type_pos{2}];%to get the runnable or AIPCALL path
      | trg_port_name = get_param(find_system(runnable_path,'BlockType','TriggerPort'),'Name');%to get the function call trigger name
      | TaskRate = '';%the raster suffix is stored in the parameter 
      | 
      | if ~isempty(trg_port_name)
      |     trg_port_name_spltd = strsplit(trg_port_name{1},'_');%splitting is done in order to get the raster and its type(Sched or Event)
      |     
      |     % checking for rasters of type Sched or Event especially occuring in
      |     % runnables
      |     if ~isempty(regexp(trg_port_name_spltd{1},'^Sched|^Event','once')) 
      |         TaskRate = ['_' regexprep(trg_port_name_spltd{1},'Sched|Event','','once')];
      |         
      |     %checking if the raster is dcmcb and this is applicable only for
      |     %APICALL
      |     elseif ~isempty(regexp([trg_port_name_spltd{1} '_' trg_port_name_spltd{2} '_' ],'^DataServices_DCM_|^RoutineServices_DCM_','once'))||...
      |             ~isempty(regexp(trg_port_name_spltd{1},'^Dcm$','once'))
      |         TaskRate = '_dcmcb';
      |         
      |     %checking if this block is used under the function call trigger
      |     %starting with "Com" and then giving an error message
      |     %this is applicable only for APICALL
      |     elseif ~isempty(regexp(trg_port_name_spltd{1},'^Com$','once'))
      |         msg = sprintf(['\n','The Supplier call block "' Thisblk '" should not be present within APICALLs having function call trigger as "Com"']);
      |         errordlg(msg);
      |         return;
      |     end
      | end
      | 
      | DataName = ['Supplier_call_ti_mini_ok_pinj3' TaskRate];%the variable name that should be given to DataStoreRead block 
      | set_param([Thisblk '/Data Store Read'],'DataStoreName',DataName);%Setting the DataStoreName of DataStoreRead block
      | 
      | %other settings done to this variable name
      | structVxx=Simulink.Signal;
      | structVxx.Dimensions=1;
      | structVxx.DimensionsMode='Fixed';
      | structVxx.DataType='boolean';
      | structVxx.Complexity='real';
      | structVxx.SamplingMode='Sample based';
      | structVxx.SampleTime=-1;
      | assignin('base',DataName,structVxx);
      settings: AttributesFormatString=%<MaskType>  RTWSystemCode=Nonreusable function  RTWFcnNameOpts=User specified
      mask Help:
      | eval('path_lib=fileparts(which(''AEMS_Standard_Library''));');
      | mskblk=get_param(gcbh,'MaskType');
      | doc_path = [path_lib '\Help\',mskblk,'.pdf'];
      | eval('open(doc_path)');
  AEMS_SUPPLIER_CALL_TI_MINI_OK_PINJ4 : Subsystem  Tag=[LIB]  TreatAsAtomicUnit=on  RTWFcnName=SUPPLIER_CALL_Ti_mini_ok_pinj4  mask(AEMS_SUPPLIER_CALL_TI_MINI_OK_PINJ4){}
      mask help:
      | Verify if the estimated fuel injection ti is over minimum possible ti.
      |
      | This block is to call Supplier call API.
      mask init:
      | Thisblk = gcb;
      | model_type_pos = strsplit(Thisblk,'/');%to split all the layer paths in order to get the runnable path
      | runnable_path = [bdroot '/' model_type_pos{2}];%to get the runnable or AIPCALL path
      | trg_port_name = get_param(find_system(runnable_path,'BlockType','TriggerPort'),'Name');%to get the function call trigger name
      | TaskRate = '';%the raster suffix is stored in the parameter 
      | 
      | if ~isempty(trg_port_name)
      |     trg_port_name_spltd = strsplit(trg_port_name{1},'_');%splitting is done in order to get the raster and its type(Sched or Event)
      |     
      |     % checking for rasters of type Sched or Event especially occuring in
      |     % runnables
      |     if ~isempty(regexp(trg_port_name_spltd{1},'^Sched|^Event','once')) 
      |         TaskRate = ['_' regexprep(trg_port_name_spltd{1},'Sched|Event','','once')];
      |         
      |     %checking if the raster is dcmcb and this is applicable only for
      |     %APICALL
      |     elseif ~isempty(regexp([trg_port_name_spltd{1} '_' trg_port_name_spltd{2} '_' ],'^DataServices_DCM_|^RoutineServices_DCM_','once'))||...
      |             ~isempty(regexp(trg_port_name_spltd{1},'^Dcm$','once'))
      |         TaskRate = '_dcmcb';
      |         
      |     %checking if this block is used under the function call trigger
      |     %starting with "Com" and then giving an error message
      |     %this is applicable only for APICALL
      |     elseif ~isempty(regexp(trg_port_name_spltd{1},'^Com$','once'))
      |         msg = sprintf(['\n','The Supplier call block "' Thisblk '" should not be present within APICALLs having function call trigger as "Com"']);
      |         errordlg(msg);
      |         return;
      |     end
      | end
      | 
      | DataName = ['Supplier_call_ti_mini_ok_pinj4' TaskRate];%the variable name that should be given to DataStoreRead block 
      | set_param([Thisblk '/DataStoreRead'],'DataStoreName',DataName);%Setting the DataStoreName of DataStoreRead block
      | 
      | %other settings done to this variable name
      | structVxx=Simulink.Signal;
      | structVxx.Dimensions=1;
      | structVxx.DimensionsMode='Fixed';
      | structVxx.DataType='boolean';
      | structVxx.Complexity='real';
      | structVxx.SamplingMode='Sample based';
      | structVxx.SampleTime=-1;
      | assignin('base',DataName,structVxx);
      settings: AttributesFormatString=%<MaskType>  RTWSystemCode=Nonreusable function  RTWFcnNameOpts=User specified
      mask Help:
      | eval('path_lib=fileparts(which(''AEMS_Standard_Library''));');
      | mskblk=get_param(gcbh,'MaskType');
      | doc_path = [path_lib '\Help\',mskblk,'.pdf'];
      | eval('open(doc_path)');
  AEMS_SUPPLIER_CALL_TI_MINI_OK_POST : Subsystem  Tag=[LIB]  TreatAsAtomicUnit=on  RTWFcnName=SUPPLIER_CALL_Ti_mini_ok_post  mask(AEMS_SUPPLIER_CALL_TI_MINI_OK_POST){}
      mask help:
      | Verify if the estimated fuel injection ti is over minimum possible ti.
      |
      | This block is to call Supplier call API.
      mask init:
      | Thisblk = gcb;
      | model_type_pos = strsplit(Thisblk,'/');%to split all the layer paths in order to get the runnable path
      | runnable_path = [bdroot '/' model_type_pos{2}];%to get the runnable or AIPCALL path
      | trg_port_name = get_param(find_system(runnable_path,'BlockType','TriggerPort'),'Name');%to get the function call trigger name
      | TaskRate = '';%the raster suffix is stored in the parameter 
      | 
      | if ~isempty(trg_port_name)
      |     trg_port_name_spltd = strsplit(trg_port_name{1},'_');%splitting is done in order to get the raster and its type(Sched or Event)
      |     
      |     % checking for rasters of type Sched or Event especially occuring in
      |     % runnables
      |     if ~isempty(regexp(trg_port_name_spltd{1},'^Sched|^Event','once')) 
      |         TaskRate = ['_' regexprep(trg_port_name_spltd{1},'Sched|Event','','once')];
      |         
      |     %checking if the raster is dcmcb and this is applicable only for
      |     %APICALL
      |     elseif ~isempty(regexp([trg_port_name_spltd{1} '_' trg_port_name_spltd{2} '_' ],'^DataServices_DCM_|^RoutineServices_DCM_','once'))||...
      |             ~isempty(regexp(trg_port_name_spltd{1},'^Dcm$','once'))
      |         TaskRate = '_dcmcb';
      |         
      |     %checking if this block is used under the function call trigger
      |     %starting with "Com" and then giving an error message
      |     %this is applicable only for APICALL
      |     elseif ~isempty(regexp(trg_port_name_spltd{1},'^Com$','once'))
      |         msg = sprintf(['\n','The Supplier call block "' Thisblk '" should not be present within APICALLs having function call trigger as "Com"']);
      |         errordlg(msg);
      |         return;
      |     end
      | end
      | 
      | DataName = ['Supplier_call_ti_mini_ok_post' TaskRate];%the variable name that should be given to DataStoreRead block 
      | set_param([Thisblk '/Data Store Read'],'DataStoreName',DataName);%Setting the DataStoreName of DataStoreRead block
      | 
      | %other settings done to this variable name
      | structVxx=Simulink.Signal;
      | structVxx.Dimensions=1;
      | structVxx.DimensionsMode='Fixed';
      | structVxx.DataType='boolean';
      | structVxx.Complexity='real';
      | structVxx.SamplingMode='Sample based';
      | structVxx.SampleTime=-1;
      | assignin('base',DataName,structVxx);
      settings: AttributesFormatString=%<MaskType>  RTWSystemCode=Nonreusable function  RTWFcnNameOpts=User specified
      mask Help:
      | eval('path_lib=fileparts(which(''AEMS_Standard_Library''));');
      | mskblk=get_param(gcbh,'MaskType');
      | doc_path = [path_lib '\Help\',mskblk,'.pdf'];
      | eval('open(doc_path)');
  AEMS_SUPPLIER_CALL_TI_MIN_OK : Subsystem  Tag=[LIB]  TreatAsAtomicUnit=on  RTWFcnName=SUPPLIER_CALL_Ti_mini_post1_ok  mask(AEMS_SUPPLIER_CALL_TI_MIN_OK){Outportname=Vbx_fms_ti_min_post2_2sl_ok, Suppliercallname=SUPPLIER_CALL_Ti_mini_post2_ok, Splitnum=2}
      mask prompts: Outportname "Outport Name"; Suppliercallname "Supplier call  Name"; Splitnum "Split"
      mask help:
      | Verify if the estimated fuel injection ti is over minimum possible ti.
      |
      | Each block will be translated into code C by this way:
      | Output=Supplier call API Name(Splitnum);
      | Example for Supplier_Call_Ti_mini_post1_ok, corresponding output variable is Vbx_fms_ti_min_post1__2sl_ok
      | Vbx_fms_ti_min_post1__2sl_ok= Supplier_Call_Ti_mini_post1_ok(1);
      mask init:
      | ThisBlk = gcb;
      | OutPorts            =   {'Vbx_fms_ti_min_post1_ok','Vbx_fms_ti_min_post1_2sl_ok','Vbx_fms_ti_min_post1_3sl_ok','Vbx_fms_ti_min_post2_2sl_ok','Vbx_fms_ti_min_post2_3sl_ok','Vbx_fms_ti_min_post3_3sl_ok'};
      | 
      | Supplier_Calls      =   {'SUPPLIER_CALL_Ti_mini_post1_ok','SUPPLIER_CALL_Ti_mini_post1_ok','SUPPLIER_CALL_Ti_mini_post1_ok','SUPPLIER_CALL_Ti_mini_post2_ok','SUPPLIER_CALL_Ti_mini_post2_ok','SUPPLIER_CALL_Ti_mini_post3_ok'};
      | 
      | Data_Names         =   {'Supplier_Call_Ti_mini_post1_ok','Supplier_Call_Ti_mini_post1_ok','Supplier_Call_Ti_mini_post1_ok','Supplier_Call_Ti_mini_post2_ok','Supplier_Call_Ti_mini_post2_ok','Supplier_Call_Ti_mini_post3_ok'};
      |                      
      | Splits              =   {'1','2','3','2','3','3'};
      | 
      | model_type_pos = strsplit(ThisBlk,'/');
      | runnable_path = [bdroot '/' model_type_pos{2}];%to get the runnable or APICALL path
      | trg_port_name = get_param(find_system(runnable_path,'BlockType','TriggerPort'),'Name');%to get the function call trigger name
      | TaskRate = '';
      | if ~isempty(trg_port_name)
      |     trg_port_name_spltd = strsplit(trg_port_name{1},'_');
      |     if ~isempty(regexp(trg_port_name_spltd{1},'^Sched|^Event','once'))
      |         TaskRate = ['_' regexprep(trg_port_name_spltd{1},'Sched|Event','','once')];
      |     elseif ~isempty(regexp([trg_port_name_spltd{1} '_' trg_port_name_spltd{2} '_' ],'^DataServices_DCM_|^RoutineServices_DCM_','once'))||...
      |             ~isempty(regexp(trg_port_name_spltd{1},'^Dcm$','once'))
      |         TaskRate = '_dcmcb';
      |     elseif ~isempty(regexp(trg_port_name_spltd{1},'^Com$','once'))
      |         msg = sprintf(['\n','The Supplier call block "' Thisblk '" should not be present within APICALLs having function call trigger as "Com"']);
      |         errordlg(msg);
      |         return;
      |     end
      | end
      | 
      | Idx_Of_Outportname = find(ismember(OutPorts,Outportname));
      | DataName = [Data_Names{Idx_Of_Outportname} TaskRate];
      | 
      | %set the  suppliername according to the Outport name.
      | set_param(ThisBlk,'Suppliercallname',Supplier_Calls{Idx_Of_Outportname});
      | set_param(ThisBlk,'Splitnum',Splits{Idx_Of_Outportname});
      | 
      | %Get the paths of the blks under this lib block.
      | Const_Blk = [ThisBlk,'/Splitnum'];%%path of "const block" inside this lib blk.
      | DSR_Blk   = [ThisBlk,'/Data_Store_Read'];%path of "Data store read block" inside this lib blk.
      | Outport_Blk = find_system(ThisBlk,'LookUnderMasks','all','FollowLinks','on','BlockType','Outport');
      | Outport_Blk = Outport_Blk{1};%I know this is d only outport blk.
      | 
      | %set the attributes of the blks under this lib block, based on teh Outportname chosen by d user.
      | set_param(Outport_Blk,'Name',Outportname);
      | set_param(DSR_Blk,'DataStoreName',DataName);
      | set_param(Const_Blk,'Value',Splits{Idx_Of_Outportname});
      | 
      | %To create a singal object in d base workspace.
      | EvalStr = ['exist(''',DataName,''',''var'')'];
      | structVxx=Simulink.Signal;
      | % structVxx=Simulink.Signal;
      | structVxx.Dimensions=1;
      | structVxx.DimensionsMode='Fixed';
      | structVxx.DataType='single';
      | structVxx.Complexity='real';
      | structVxx.SamplingMode='Sample based';
      | structVxx.SampleTime=-1;
      | isDefined= evalin('base',EvalStr);%This line checks whether the DataName exist in the base workspace.
      | if (isDefined==0)
      |     assignin('base',DataName,structVxx);
      | end
      settings: RTWSystemCode=Inline  RTWFcnNameOpts=User specified
      settings: AttributesFormatString=|
      | %<MaskType>
      | Outport Name = %<Outportname>
      | Supplier Call Name = %<Suppliercallname>
      | Split number = %<Splitnum>
      mask Help:
      | eval('path_lib=fileparts(which(''AEMS_Standard_Library''));');
      | mskblk=get_param(gcbh,'MaskType');
      | doc_path = [path_lib '\Help\',mskblk,'.pdf'];
      | eval('open(doc_path)');
      mask TypeOptions Outportname: Vbx_fms_ti_min_post1_ok | Vbx_fms_ti_min_post1_2sl_ok | Vbx_fms_ti_min_post1_3sl_ok | Vbx_fms_ti_min_post2_2sl_ok | Vbx_fms_ti_min_post2_3sl_ok | Vbx_fms_ti_min_post3_3sl_ok
      mask Callback Outportname:
      | OutPorts            =   {'Vbx_fms_ti_min_post1_ok','Vbx_fms_ti_min_post1_2sl_ok','Vbx_fms_ti_min_post1_3sl_ok','Vbx_fms_ti_min_post2_2sl_ok','Vbx_fms_ti_min_post2_3sl_ok','Vbx_fms_ti_min_post3_3sl_ok'};
      | 
      | Supplier_Calls      =   {'SUPPLIER_CALL_Ti_mini_post1_ok','SUPPLIER_CALL_Ti_mini_post1_ok','SUPPLIER_CALL_Ti_mini_post1_ok','SUPPLIER_CALL_Ti_mini_post2_ok','SUPPLIER_CALL_Ti_mini_post2_ok','SUPPLIER_CALL_Ti_mini_post3_ok'};
      | 
      | Splits              =   {'1','2','3','2','3','3'};
      | 
      | 
      | Outportname = get_param(gcb,'Outportname');
      | 
      | Idx_Of_Outportname = find(ismember(OutPorts,Outportname));
      | %set the  suppliername according to the Outport name.
      | set_param(gcb,'Suppliercallname',Supplier_Calls{Idx_Of_Outportname});
      | set_param(gcb,'Splitnum',Splits{Idx_Of_Outportname});
      | 
      | cellfun(@clear,{'Idx_Of_Outportname','Outportname','OutPorts','Splits','Supplier_Calls'});
  AEMS_SlopeSwitchExtern : Subsystem  Tag=[LIB]  mask(AEMS_SlopeSwitchExtern){LimitDimInputs=2, Indexmode=Zero-based}
      mask prompts: LimitDimInputs "Limit of Input Dimension"; Indexmode "Index Mode for Switch Port"
      mask help:
      | This block is a Multiple Port Slope Switch.
      | Depending on the value of input Switch_Cmd (from 0), the block outputs the corresponding input signal.
      | For Switch_Cmd = 0, Output is In0, for Switch_Cmd = 1, Output is In1, and so on...
      |
      | Nevertheless, for each switch between two input signals, a slope is activated from the first input signal to the second input signal.
      | The value of this slope is given by Pos_Slope if the input signal to reach is over the initial input signal and by Neg_Slope if the input signal to reach is under.
      | Pos_Slope and Neg_Slope are respectively the positive and negative slope parameters per second.
      |
      | The output Slope_On indicates if a transition is active (Slope_On at true) or not (Slope_On at false).
      mask init:
      | set_param([get_param(gcb,'Parent'),'/',get_param(gcb,'Name'),'/Selector'],'IndexMode',Indexmode);
      | 
      | if strcmp(Indexmode,'Zero-based')
      |     idx_val = 1;
      | else
      |     idx_val = 2;
      | end
      | 
      | up_limit = LimitDimInputs+idx_val-2;
      | low_limit = idx_val-1;
      | 
      | set_param([gcb,'/Saturation'],'UpperLimit',num2str(LimitDimInputs+idx_val-2));
      | set_param([gcb,'/Saturation'],'LowerLimit',num2str(idx_val-1));
      settings: AttributesFormatString=|
      | %<MaskType>
      | Limit of Input Dimension: %<LimitDimInputs>
      | Switch Index mode: %<Indexmode>
      mask Help:
      | eval('path_lib=fileparts(which(''AEMS_Standard_Library''));');
      | mskblk=get_param(gcbh,'MaskType');
      | doc_path = [path_lib '\Help\',mskblk,'.pdf'];
      | eval('open(doc_path)');
      mask TypeOptions Indexmode: Zero-based | One-based
      mask Display:
      | color ('blue')
      | disp('SLOPE \n\n SWITCH EXTERN')
  AEMS_UL_INTERP : Subsystem  Tag=[LIB]  Description=This library calculates interpolation for 2 inputs.  mask(AEMS_UL_INTERP){}
      mask help:
      | Interpolation for 2inputs
      |
      | output = input_of_ratio_1 * interpolate_ratio
      |          + input_of_ratio_0 * ( 1 - interpolate_ratio )
      |
      | I/O
      |     input_of_ratio_1
      |         Input of ratio term
      |     input_of_ratio_0
      |         Input of 1 - ratio term
      |     interpolate_ratio
      |         Interpolate Ratio ( 0 <= interpolate_ratio <= 1 )
      |
      | output
      |         Output value
      settings: AttributesFormatString=%<MaskType>
      mask Help:
      | eval('path_lib=fileparts(which(''AEMS_Standard_Library''));');
      | doc_path = [path_lib '\help\AEMS_UL_INTERP.pdf'];
      | eval('open(doc_path)')
      mask Display: disp('AEMS_UL_INTERP')
